simulink model "ICAR"  (R2018b)
settings: Solver=FixedStepAuto  StartTime=0.0  StopTime=10.0  RelTol=1e-3
(part 3 of 4)

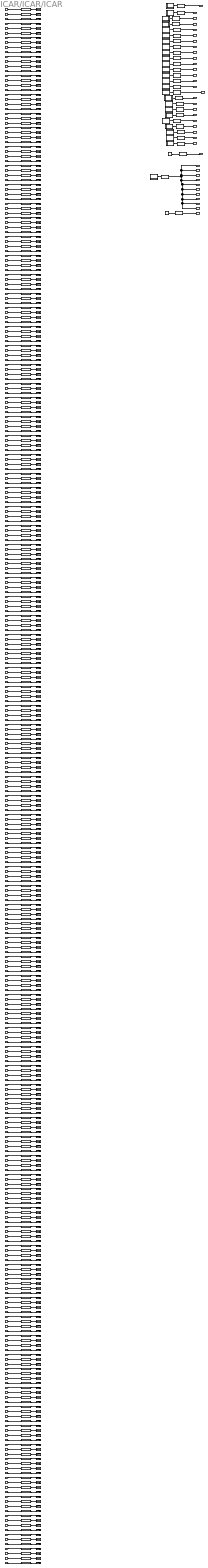
== system ICAR/ICAR/ICAR ==
  System_Clock : Inport  OutDataTypeStr=UInt16
  FDMMve_d_IcaFcnConf : Inport  Port=2  OutDataTypeStr=UInt16
  FDMMve_d_SignalTStamp : Inport  Port=3  OutDataTypeStr=UInt16
  ICABva_g_VehParameter : Inport  Port=4  OutDataTypeStr=T_M_Nm_Float32  PortDimensions=60
  ICABva_g_FilterInfo : Inport  Port=5  OutDataTypeStr=T_M_Nm_Float32  PortDimensions=50
  ICABve_d_SignalTStamp : Inport  Port=6  OutDataTypeStr=UInt16
  IMAPve_d_EPS_LKA_State : Inport  Port=7  OutDataTypeStr=UInt16
  IMAPve_g_EPS_SW_Trq : Inport  Port=8  OutDataTypeStr=T_M_Nm_Float32
  IMAPve_d_EPS_Error_State : Inport  Port=9  OutDataTypeStr=UInt16
  IMAPve_d_EPS_Trq_State : Inport  Port=10  OutDataTypeStr=UInt16
  IMAPve_d_SAS_Clb_State : Inport  Port=11  OutDataTypeStr=UInt16
  IMAPve_d_SAS_Trim_State : Inport  Port=12  OutDataTypeStr=UInt16
  IMAPve_d_EPS_TrqLim_State : Inport  Port=13  OutDataTypeStr=UInt16
  IMAPve_g_EPS_LKA_Current : Inport  Port=14  OutDataTypeStr=T_M_Nm_Float32
  IMAPve_g_ESC_LatAcc : Inport  Port=15  OutDataTypeStr=T_M_Nm_Float32
  IMAPve_d_ESC_LatAcc_Valid : Inport  Port=16  OutDataTypeStr=UInt16
  IMAPve_g_ESC_YawRate : Inport  Port=17  OutDataTypeStr=T_M_Nm_Float32
  IMAPve_d_ESC_YawRate_Valid : Inport  Port=18  OutDataTypeStr=UInt16
  IMAPve_g_ESC_UnYawRate : Inport  Port=19  OutDataTypeStr=T_M_Nm_Float32
  IMAPve_g_ESC_VehSpd : Inport  Port=20  OutDataTypeStr=T_M_Nm_Float32
  IMAPve_g_ESC_LonAcc : Inport  Port=21  OutDataTypeStr=T_M_Nm_Float32
  IMAPve_d_ESC_LonAcc_Valid : Inport  Port=22  OutDataTypeStr=UInt16
  IMAPve_g_ESC_Brake_Press : Inport  Port=23  OutDataTypeStr=T_M_Nm_Float32
  IMAPve_g_ESC_Static_Slope : Inport  Port=24  OutDataTypeStr=T_M_Nm_Float32
  IMAPve_g_ESC_DySlope_Accuracy : Inport  Port=25  OutDataTypeStr=T_M_Nm_Float32
  IMAPve_g_ESC_DySlope : Inport  Port=26  OutDataTypeStr=T_M_Nm_Float32
  IMAPve_g_SW_Angle : Inport  Port=27  OutDataTypeStr=T_M_Nm_Float32
  IMAPve_g_SW_Angle_Speed : Inport  Port=28  OutDataTypeStr=T_M_Nm_Float32
  IMAPve_d_BCM_HazardLamp : Inport  Port=29  OutDataTypeStr=UInt16
  IMAPve_d_BCM_Left_Light : Inport  Port=30  OutDataTypeStr=UInt16
  IMAPve_d_BCM_Right_Light : Inport  Port=31  OutDataTypeStr=UInt16
  IMAPve_d_ESC_BrakeLamp_Req : Inport  Port=32  OutDataTypeStr=UInt16
  IMAPve_d_BCM_Opening_State : Inport  Port=33  OutDataTypeStr=UInt16
  IMAPve_d_BCM_Trunk_State : Inport  Port=34  OutDataTypeStr=UInt16
  IMAPve_d_BCM_LF_Door_State : Inport  Port=35  OutDataTypeStr=UInt16
  IMAPve_d_BCM_RF_Door_State : Inport  Port=36  OutDataTypeStr=UInt16
  IMAPve_d_BCM_RR_Door_State : Inport  Port=37  OutDataTypeStr=UInt16
  IMAPve_d_BCM_LR_Door_State : Inport  Port=38  OutDataTypeStr=UInt16
  IMAPve_d_SCC_Left_SwitchSig : Inport  Port=39  OutDataTypeStr=UInt16
  IMAPve_d_SCC_Right_SwitchSig : Inport  Port=40  OutDataTypeStr=UInt16
  IMAPve_d_PEPS_Door_Lock_Req : Inport  Port=41  OutDataTypeStr=UInt16
  IMAPve_d_BCM_Door_Lock_State : Inport  Port=42  OutDataTypeStr=UInt16
  IMAPve_d_EMS_ACC_Status : Inport  Port=43  OutDataTypeStr=UInt16
  IMAPve_g_EMS_Pot_WhlT_Max : Inport  Port=44  OutDataTypeStr=T_M_Nm_Float32
  IMAPve_g_EMS_Pot_WhlT_Min : Inport  Port=45  OutDataTypeStr=T_M_Nm_Float32
  IMAPve_g_EMS_RealPedal : Inport  Port=46  OutDataTypeStr=T_M_Nm_Float32
  IMAPve_g_EMS_MaxTWhl : Inport  Port=47  OutDataTypeStr=T_M_Nm_Float32
  IMAPve_g_EMS_MaxTWhl_Offset : Inport  Port=48  OutDataTypeStr=T_M_Nm_Float32
  IMAPve_g_EMS_MinTWhl : Inport  Port=49  OutDataTypeStr=T_M_Nm_Float32
  IMAPve_g_EMS_MinTWhl_Offset : Inport  Port=50  OutDataTypeStr=T_M_Nm_Float32
  IMAPve_g_EMS_Actual_FlwT : Inport  Port=51  OutDataTypeStr=T_M_Nm_Float32
  IMAPve_g_EMS_Actual_IndT : Inport  Port=52  OutDataTypeStr=T_M_Nm_Float32
  IMAPve_g_EMS_Realize_TWhl : Inport  Port=53  OutDataTypeStr=T_M_Nm_Float32
  IMAPve_g_EMS_ACC_VirtualPedal : Inport  Port=54  OutDataTypeStr=T_M_Nm_Float32
  IMAPve_d_EMS_AccPedal_Fault : Inport  Port=55  OutDataTypeStr=UInt16
  IMAPve_g_EMS_Driver_Torque : Inport  Port=56  OutDataTypeStr=T_M_Nm_Float32
  IMAPve_d_ESC_Brake_Effort : Inport  Port=57  OutDataTypeStr=UInt16
  IMAPve_g_EMS_Engine_Speed : Inport  Port=58  OutDataTypeStr=T_M_Nm_Float32
  IMAPve_d_ESC_Veh_Standstill : Inport  Port=59  OutDataTypeStr=UInt16
  IMAPve_d_TCU_Actual_Gear : Inport  Port=60  OutDataTypeStr=UInt16
  IMAPve_d_TCU_Target_Gear : Inport  Port=61  OutDataTypeStr=UInt16
  IMAPve_d_TCU_PRND_State : Inport  Port=62  OutDataTypeStr=UInt16
  IMAPve_d_BCM_Ignition_State : Inport  Port=63  OutDataTypeStr=UInt16
  IMAPve_d_ACU_Driver_Belt : Inport  Port=64  OutDataTypeStr=UInt16
  IMAPve_d_SWS_Fault_Code : Inport  Port=65  OutDataTypeStr=UInt16
  IMAPve_d_SWS_Failure_Status : Inport  Port=66  OutDataTypeStr=UInt16
  IMAPve_d_ESC_OFF : Inport  Port=67  OutDataTypeStr=UInt16
  IMAPve_d_ESC_AlarmSig : Inport  Port=68  OutDataTypeStr=UInt16
  IMAPve_d_Speed_Limit_Switch : Inport  Port=69  OutDataTypeStr=UInt16
  IMAPve_d_ESC_ESC_Active : Inport  Port=70  OutDataTypeStr=UInt16
  IMAPve_d_ESC_MSR_Active : Inport  Port=71  OutDataTypeStr=UInt16
  IMAPve_d_ESC_TCS_Active : Inport  Port=72  OutDataTypeStr=UInt16
  IMAPve_d_ESC_VehSpd_Valid : Inport  Port=73  OutDataTypeStr=UInt16
  IMAPve_d_Brake_Pedal_Fault : Inport  Port=74  OutDataTypeStr=UInt16
  IMAPve_d_ESC_ABS_Active : Inport  Port=75  OutDataTypeStr=UInt16
  IMAPve_d_ESC_ABS_Valid : Inport  Port=76  OutDataTypeStr=UInt16
  IMAPve_d_ESC_ABS_AlarmSig : Inport  Port=77  OutDataTypeStr=UInt16
  IMAPve_d_ESC_FL_WheelPulVal : Inport  Port=78  OutDataTypeStr=UInt16
  IMAPve_d_ESC_FR_WheelPulVal : Inport  Port=79  OutDataTypeStr=UInt16
  IMAPve_d_ESC_RL_WheelPulVal : Inport  Port=80  OutDataTypeStr=UInt16
  IMAPve_d_ESC_RR_WheelPulVal : Inport  Port=81  OutDataTypeStr=UInt16
  IMAPve_g_ESC_FL_WhlSpd : Inport  Port=82  OutDataTypeStr=T_M_Nm_Float32
  IMAPve_d_ESC_FL_WhlSpd_Fault : Inport  Port=83  OutDataTypeStr=UInt16
  IMAPve_g_ESC_FR_WhlSpd : Inport  Port=84  OutDataTypeStr=T_M_Nm_Float32
  IMAPve_d_ESC_FR_WhlSpd_Fault : Inport  Port=85  OutDataTypeStr=UInt16
  IMAPve_g_ESC_RL_WhlSpd : Inport  Port=86  OutDataTypeStr=T_M_Nm_Float32
  IMAPve_d_ESC_RL_WhlSpd_Fault : Inport  Port=87  OutDataTypeStr=UInt16
  IMAPve_g_ESC_RR_WhlSpd : Inport  Port=88  OutDataTypeStr=T_M_Nm_Float32
  IMAPve_d_ESC_RR_WhlSpd_Fault : Inport  Port=89  OutDataTypeStr=UInt16
  IMAPve_d_ESC_FL_Wheel_Pulse : Inport  Port=90  OutDataTypeStr=UInt16
  IMAPve_d_ESC_FR_Wheel_Pulse : Inport  Port=91  OutDataTypeStr=UInt16
  IMAPve_d_ESC_RL_Wheel_Pulse : Inport  Port=92  OutDataTypeStr=UInt16
  IMAPve_d_ESC_RR_Wheel_Pulse : Inport  Port=93  OutDataTypeStr=UInt16
  IMAPve_d_TCU_AT_Failure : Inport  Port=94  OutDataTypeStr=UInt16
  IMAPve_d_TCU_Shift_Valid : Inport  Port=95  OutDataTypeStr=UInt16
  IMAPve_d_TCU_DCT_Clutch_State : Inport  Port=96  OutDataTypeStr=UInt16
  IMAPve_d_TCU_Gear_Engage : Inport  Port=97  OutDataTypeStr=UInt16
  IMAPve_d_TCU_Select_ATMode : Inport  Port=98  OutDataTypeStr=UInt16
  IMAPve_d_EMS_Engine_Status : Inport  Port=99  OutDataTypeStr=UInt16
  IMAPve_d_EMS_Gearbox_CtlAvail : Inport  Port=100  OutDataTypeStr=UInt16
  IMAPve_d_ESC_Brake_Failsafe : Inport  Port=101  OutDataTypeStr=UInt16
  IMAPve_d_ESC_AEB_Status : Inport  Port=102  OutDataTypeStr=UInt16
  IMAPve_d_ESC_AEB_Available : Inport  Port=103  OutDataTypeStr=UInt16
  IMAPve_d_ESC_AEB_Active : Inport  Port=104  OutDataTypeStr=UInt16
  IMAPve_d_ESC_ACC_Status : Inport  Port=105  OutDataTypeStr=UInt16
  IMAPve_d_ESC_ACC_Available : Inport  Port=106  OutDataTypeStr=UInt16
  IMAPve_d_ESC_ACC_Active : Inport  Port=107  OutDataTypeStr=UInt16
  IMAPve_d_EMS_ACC_Effective : Inport  Port=108  OutDataTypeStr=UInt16
  IMAPve_d_BCM_FrontWiper_State : Inport  Port=109  OutDataTypeStr=UInt16
  IMAPve_d_BCM_CHMSL_Status : Inport  Port=110  OutDataTypeStr=UInt16
  IMAPve_d_BCM_BrakeLamp_State : Inport  Port=111  OutDataTypeStr=UInt16
  IMAPve_d_GW_Brake_Only_Req : Inport  Port=112  OutDataTypeStr=UInt16
  IMAPve_d_ACU_Passenger_Belt : Inport  Port=113  OutDataTypeStr=UInt16
  IMAPve_d_EMS_ACC_CtlAvail : Inport  Port=114  OutDataTypeStr=UInt16
  IMAPve_d_EMS_ACC_Inhibited : Inport  Port=115  OutDataTypeStr=UInt16
  IMAPve_d_EMS_Brake_Pedal : Inport  Port=116  OutDataTypeStr=UInt16
  IMAPve_d_BCM_LowBeam_State : Inport  Port=117  OutDataTypeStr=UInt16
  IMAPve_d_BCM_HighBeam_State : Inport  Port=118  OutDataTypeStr=UInt16
  IMAPve_d_EPB_Status : Inport  Port=119  OutDataTypeStr=UInt16
  IMAPve_d_EPB_Display_Req : Inport  Port=120  OutDataTypeStr=UInt16
  IMAPve_d_EPB_Warn_Req : Inport  Port=121  OutDataTypeStr=UInt16
  IMAPve_d_EPB_Switch_State : Inport  Port=122  OutDataTypeStr=UInt16
  IMAPve_d_EPB_Switch_Valid : Inport  Port=123  OutDataTypeStr=UInt16
  IMAPve_d_ESC_Drive_Direction : Inport  Port=124  OutDataTypeStr=UInt16
  IMAPve_d_ESC_Hold_State : Inport  Port=125  OutDataTypeStr=UInt16
  IMAPve_d_EPS_Steer_Hold_State : Inport  Port=126  OutDataTypeStr=UInt16
  IMAPve_d_EPS_Warning_State : Inport  Port=127  OutDataTypeStr=UInt16
  IMAPve_g_EPS_PowerCon : Inport  Port=128  OutDataTypeStr=T_M_Nm_Float32
  IMAPve_d_ESC_EBD_AlarmSig : Inport  Port=129  OutDataTypeStr=UInt16
  IMAPve_d_ESC_AVH_Status : Inport  Port=130  OutDataTypeStr=UInt16
  IMAPve_d_Radar_Detective_Req : Inport  Port=131  OutDataTypeStr=UInt16
  IMAPve_g_BCM_Battery_Voltage : Inport  Port=132  OutDataTypeStr=T_M_Nm_Float32
  IMAPve_d_TBOX_LocalTimeY : Inport  Port=133  OutDataTypeStr=UInt16
  IMAPve_d_TBOX_LocalTimeM : Inport  Port=134  OutDataTypeStr=UInt16
  IMAPve_d_TBOX_LocalTimeD : Inport  Port=135  OutDataTypeStr=UInt16
  IMAPve_d_TBOX_LocalTimeH : Inport  Port=136  OutDataTypeStr=UInt16
  IMAPve_d_TBOX_LocalTimeMin : Inport  Port=137  OutDataTypeStr=UInt16
  IMAPve_d_TBOX_LocalTimeS : Inport  Port=138  OutDataTypeStr=UInt16
  IMAPve_d_TBOX_LocalTime_Valid : Inport  Port=139  OutDataTypeStr=UInt16
  IMAPve_d_TPMS_Warn_Indicate : Inport  Port=140  OutDataTypeStr=UInt16
  IMAPve_d_Radar_State : Inport  Port=141  OutDataTypeStr=UInt16
  IMAPve_d_ACC_Desired_Headway : Inport  Port=142  OutDataTypeStr=UInt16
  IMAPve_d_Time_System_Clock : Inport  Port=143  OutDataTypeStr=UInt16
  IMAPve_d_Signal_Time_Stamp : Inport  Port=144  OutDataTypeStr=UInt16
  IMAPve_g_GW_IC_Odometer : Inport  Port=145  OutDataTypeStr=UInt32
  IMAPve_g_FAPA_State : Inport  Port=146  OutDataTypeStr=UInt32
  IMAPve_d_Outside_Temp : Inport  Port=147  OutDataTypeStr=UInt16
  IMAPve_d_ORI_CIPV_ID : Inport  Port=148  OutDataTypeStr=UInt16
  IMAPve_d_ORI_Obj_Num : Inport  Port=149  OutDataTypeStr=UInt16
  IMAPva_g_ORI_Probability : Inport  Port=150  OutDataTypeStr=T_M_Nm_Float32  PortDimensions=16
  IMAPva_d_ORI_Obj_Class : Inport  Port=151  OutDataTypeStr=UInt16  PortDimensions=16
  IMAPva_d_ORI_Obj_Motion : Inport  Port=152  OutDataTypeStr=UInt16  PortDimensions=16
  IMAPva_g_ORI_Obj_RelVel : Inport  Port=153  OutDataTypeStr=T_M_Nm_Float32  PortDimensions=16
  IMAPva_g_ORI_Obj_LongDis : Inport  Port=154  OutDataTypeStr=T_M_Nm_Float32  PortDimensions=16
  IMAPva_d_ORI_Obj_Lane : Inport  Port=155  OutDataTypeStr=UInt16  PortDimensions=16
  IMAPva_g_ORI_Obj_LAngle : Inport  Port=156  OutDataTypeStr=T_M_Nm_Float32  PortDimensions=16
  IMAPva_g_ORI_Obj_RAngle : Inport  Port=157  OutDataTypeStr=T_M_Nm_Float32  PortDimensions=16
  IMAPva_g_ORI_Obj_Width : Inport  Port=158  OutDataTypeStr=T_M_Nm_Float32  PortDimensions=16
  IMAPva_d_ORI_Obj_ID : Inport  Port=159  OutDataTypeStr=UInt16  PortDimensions=16
  IMAPve_d_ORI_Lane_Valid : Inport  Port=160  OutDataTypeStr=UInt16
  IMAPve_d_ORI_Lane_ConsArea : Inport  Port=161  OutDataTypeStr=UInt16
  IMAPve_d_ORI_Lane_RoadType : Inport  Port=162  OutDataTypeStr=UInt16
  IMAPve_g_ORI_L0_C3 : Inport  Port=163  OutDataTypeStr=T_M_Nm_Float32
  IMAPve_g_ORI_L0_C2 : Inport  Port=164  OutDataTypeStr=T_M_Nm_Float32
  IMAPve_g_ORI_L0_C1 : Inport  Port=165  OutDataTypeStr=T_M_Nm_Float32
  IMAPve_g_ORI_L0_C0 : Inport  Port=166  OutDataTypeStr=T_M_Nm_Float32
  IMAPve_d_ORI_L0_Q : Inport  Port=167  OutDataTypeStr=UInt16
  IMAPve_d_ORI_L0_Type : Inport  Port=168  OutDataTypeStr=UInt16
  IMAPve_g_ORI_L0_VR : Inport  Port=169  OutDataTypeStr=T_M_Nm_Float32
  IMAPve_g_ORI_L0_TLC : Inport  Port=170  OutDataTypeStr=T_M_Nm_Float32
  IMAPve_g_ORI_L0_W : Inport  Port=171  OutDataTypeStr=T_M_Nm_Float32
  IMAPve_d_ORI_L0_LC : Inport  Port=172  OutDataTypeStr=UInt16
  IMAPve_g_ORI_L1_C3 : Inport  Port=173  OutDataTypeStr=T_M_Nm_Float32
  IMAPve_g_ORI_L1_C2 : Inport  Port=174  OutDataTypeStr=T_M_Nm_Float32
  IMAPve_g_ORI_L1_C1 : Inport  Port=175  OutDataTypeStr=T_M_Nm_Float32
  IMAPve_g_ORI_L1_C0 : Inport  Port=176  OutDataTypeStr=T_M_Nm_Float32
  IMAPve_d_ORI_L1_Q : Inport  Port=177  OutDataTypeStr=UInt16
  IMAPve_d_ORI_L1_Type : Inport  Port=178  OutDataTypeStr=UInt16
  IMAPve_g_ORI_L1_VR : Inport  Port=179  OutDataTypeStr=T_M_Nm_Float32
  IMAPve_g_ORI_L1_TLC : Inport  Port=180  OutDataTypeStr=T_M_Nm_Float32
  IMAPve_g_ORI_L1_W : Inport  Port=181  OutDataTypeStr=T_M_Nm_Float32
  IMAPve_d_ORI_L1_LC : Inport  Port=182  OutDataTypeStr=UInt16
  IMAPve_g_ORI_R0_C3 : Inport  Port=183  OutDataTypeStr=T_M_Nm_Float32
  IMAPve_g_ORI_R0_C2 : Inport  Port=184  OutDataTypeStr=T_M_Nm_Float32
  IMAPve_g_ORI_R0_C1 : Inport  Port=185  OutDataTypeStr=T_M_Nm_Float32
  IMAPve_g_ORI_R0_C0 : Inport  Port=186  OutDataTypeStr=T_M_Nm_Float32
  IMAPve_d_ORI_R0_Q : Inport  Port=187  OutDataTypeStr=UInt16
  IMAPve_d_ORI_R0_LT : Inport  Port=188  OutDataTypeStr=UInt16
  IMAPve_g_ORI_R0_VR : Inport  Port=189  OutDataTypeStr=T_M_Nm_Float32
  IMAPve_g_ORI_R0_TLC : Inport  Port=190  OutDataTypeStr=T_M_Nm_Float32
  IMAPve_g_ORI_R0_W : Inport  Port=191  OutDataTypeStr=T_M_Nm_Float32
  IMAPve_d_ORI_R0_LC : Inport  Port=192  OutDataTypeStr=UInt16
  IMAPve_g_ORI_R1_C3 : Inport  Port=193  OutDataTypeStr=T_M_Nm_Float32
  IMAPve_g_ORI_R1_C2 : Inport  Port=194  OutDataTypeStr=T_M_Nm_Float32
  IMAPve_g_ORI_R1_C1 : Inport  Port=195  OutDataTypeStr=T_M_Nm_Float32
  IMAPve_g_ORI_R1_C0 : Inport  Port=196  OutDataTypeStr=T_M_Nm_Float32
  IMAPve_d_ORI_R1_Q : Inport  Port=197  OutDataTypeStr=UInt16
  IMAPve_d_ORI_R1_LT : Inport  Port=198  OutDataTypeStr=UInt16
  IMAPve_g_ORI_R1_VR : Inport  Port=199  OutDataTypeStr=T_M_Nm_Float32
  IMAPve_g_ORI_R1_TLC : Inport  Port=200  OutDataTypeStr=T_M_Nm_Float32
  IMAPve_g_ORI_R1_W : Inport  Port=201  OutDataTypeStr=T_M_Nm_Float32
  IMAPve_d_ORI_R1_LC : Inport  Port=202  OutDataTypeStr=UInt16
  IMAPve_d_Sensor_Status : Inport  Port=203  OutDataTypeStr=UInt16
  IMAPve_d_LF_Radar_Status : Inport  Port=204  OutDataTypeStr=UInt16
  IMAPve_d_RF_Radar_Status : Inport  Port=205  OutDataTypeStr=UInt16
  IMAPve_d_LR_Radar_Status : Inport  Port=206  OutDataTypeStr=UInt16
  IMAPve_d_RR_Radar_Status : Inport  Port=207  OutDataTypeStr=UInt16
  IMAPve_d_Fusion_Status : Inport  Port=208  OutDataTypeStr=UInt16
  IMAPve_g_Fusion_Time_Stamp : Inport  Port=209  OutDataTypeStr=T_M_Nm_Float32
  IMAPve_d_obj_Num : Inport  Port=210  OutDataTypeStr=UInt16
  IMAPva_d_obj_id : Inport  Port=211  OutDataTypeStr=UInt16  PortDimensions=40
  IMAPva_g_obj_pos_x : Inport  Port=212  OutDataTypeStr=T_M_Nm_Float32  PortDimensions=40
  IMAPva_g_obj_pos_y : Inport  Port=213  OutDataTypeStr=T_M_Nm_Float32  PortDimensions=40
  IMAPva_g_obj_vel_x : Inport  Port=214  OutDataTypeStr=T_M_Nm_Float32  PortDimensions=40
  IMAPva_g_obj_vel_y : Inport  Port=215  OutDataTypeStr=T_M_Nm_Float32  PortDimensions=40
  IMAPva_g_obj_acc_x : Inport  Port=216  OutDataTypeStr=T_M_Nm_Float32  PortDimensions=40
  IMAPva_g_obj_acc_y : Inport  Port=217  OutDataTypeStr=T_M_Nm_Float32  PortDimensions=40
  IMAPva_g_obj_pos_var_x : Inport  Port=218  OutDataTypeStr=T_M_Nm_Float32  PortDimensions=40
  IMAPva_g_obj_pos_var_y : Inport  Port=219  OutDataTypeStr=T_M_Nm_Float32  PortDimensions=40
  IMAPva_g_obj_pos_var_xy : Inport  Port=220  OutDataTypeStr=T_M_Nm_Float32  PortDimensions=40
  IMAPva_g_obj_vel_var_x : Inport  Port=221  OutDataTypeStr=T_M_Nm_Float32  PortDimensions=40
  IMAPva_g_obj_vel_var_y : Inport  Port=222  OutDataTypeStr=T_M_Nm_Float32  PortDimensions=40
  IMAPva_g_obj_vel_var_xy : Inport  Port=223  OutDataTypeStr=T_M_Nm_Float32  PortDimensions=40
  IMAPva_g_obj_width : Inport  Port=224  OutDataTypeStr=T_M_Nm_Float32  PortDimensions=40
  IMAPva_g_obj_length : Inport  Port=225  OutDataTypeStr=T_M_Nm_Float32  PortDimensions=40
  IMAPva_d_obj_fusion_type : Inport  Port=226  OutDataTypeStr=UInt16  PortDimensions=40
  IMAPva_d_obj_class : Inport  Port=227  OutDataTypeStr=UInt16  PortDimensions=40
  IMAPva_d_obj_lane : Inport  Port=228  OutDataTypeStr=UInt16  PortDimensions=40
  IMAPva_d_obj_status : Inport  Port=229  OutDataTypeStr=UInt16  PortDimensions=40
  IMAPva_d_obj_cam_asso_id : Inport  Port=230  OutDataTypeStr=UInt16  PortDimensions=40
  IMAPva_g_obj_con : Inport  Port=231  OutDataTypeStr=T_M_Nm_Float32  PortDimensions=40
  IMAPva_g_obj_age : Inport  Port=232  OutDataTypeStr=T_M_Nm_Float32  PortDimensions=40
  IMAPva_d_obj_TurnLight : Inport  Port=233  OutDataTypeStr=UInt16  PortDimensions=40
  IMAPva_d_obj_BrakeLight : Inport  Port=234  OutDataTypeStr=UInt16  PortDimensions=40
  IMAPva_d_obj_MotionStatus : Inport  Port=235  OutDataTypeStr=UInt16  PortDimensions=40
  IMAPva_d_obj_ACC : Inport  Port=236  OutDataTypeStr=UInt16  PortDimensions=40
  IMAPva_d_obj_AEB : Inport  Port=237  OutDataTypeStr=UInt16  PortDimensions=40
  IMAPva_d_obj_ELK : Inport  Port=238  OutDataTypeStr=UInt16  PortDimensions=40
  IMAPva_d_obj_ALC : Inport  Port=239  OutDataTypeStr=UInt16  PortDimensions=40
  IMAPva_d_obj_ESA : Inport  Port=240  OutDataTypeStr=UInt16  PortDimensions=40
  IMAPva_d_obj_JA : Inport  Port=241  OutDataTypeStr=UInt16  PortDimensions=40
  IMAPve_d_Lane_Valid : Inport  Port=242  OutDataTypeStr=UInt16
  IMAPve_d_Road_Type : Inport  Port=243  OutDataTypeStr=UInt16
  IMAPve_d_ConsArea : Inport  Port=244  OutDataTypeStr=UInt16
  IMAPve_g_L0_C0 : Inport  Port=245  OutDataTypeStr=T_M_Nm_Float32
  IMAPve_g_L0_C1 : Inport  Port=246  OutDataTypeStr=T_M_Nm_Float32
  IMAPve_g_L0_C2 : Inport  Port=247  OutDataTypeStr=T_M_Nm_Float32
  IMAPve_g_L0_C3 : Inport  Port=248  OutDataTypeStr=T_M_Nm_Float32
  IMAPve_g_L0_VR : Inport  Port=249  OutDataTypeStr=T_M_Nm_Float32
  IMAPve_d_L0_Q : Inport  Port=250  OutDataTypeStr=UInt16
  IMAPve_d_L0_Type : Inport  Port=251  OutDataTypeStr=UInt16
  IMAPve_g_L0_Confidence : Inport  Port=252  OutDataTypeStr=T_M_Nm_Float32
  IMAPve_g_L0_W : Inport  Port=253  OutDataTypeStr=T_M_Nm_Float32
  IMAPve_g_L0_TLC : Inport  Port=254  OutDataTypeStr=T_M_Nm_Float32
  IMAPve_d_L0_LC : Inport  Port=255  OutDataTypeStr=UInt16
  IMAPve_g_R0_C0 : Inport  Port=256  OutDataTypeStr=T_M_Nm_Float32
  IMAPve_g_R0_C1 : Inport  Port=257  OutDataTypeStr=T_M_Nm_Float32
  IMAPve_g_R0_C2 : Inport  Port=258  OutDataTypeStr=T_M_Nm_Float32
  IMAPve_g_R0_C3 : Inport  Port=259  OutDataTypeStr=T_M_Nm_Float32
  IMAPve_g_R0_VR : Inport  Port=260  OutDataTypeStr=T_M_Nm_Float32
  IMAPve_d_R0_Q : Inport  Port=261  OutDataTypeStr=UInt16
  IMAPve_d_R0_Type : Inport  Port=262  OutDataTypeStr=UInt16
  IMAPve_g_R0_Confidence : Inport  Port=263  OutDataTypeStr=T_M_Nm_Float32
  IMAPve_g_R0_W : Inport  Port=264  OutDataTypeStr=T_M_Nm_Float32
  IMAPve_g_R0_TLC : Inport  Port=265  OutDataTypeStr=T_M_Nm_Float32
  IMAPve_d_R0_LC : Inport  Port=266  OutDataTypeStr=UInt16
  IMAPve_g_L1_C0 : Inport  Port=267  OutDataTypeStr=T_M_Nm_Float32
  IMAPve_g_L1_C1 : Inport  Port=268  OutDataTypeStr=T_M_Nm_Float32
  IMAPve_g_L1_C2 : Inport  Port=269  OutDataTypeStr=T_M_Nm_Float32
  IMAPve_g_L1_C3 : Inport  Port=270  OutDataTypeStr=T_M_Nm_Float32
  IMAPve_g_L1_VR : Inport  Port=271  OutDataTypeStr=T_M_Nm_Float32
  IMAPve_d_L1_Q : Inport  Port=272  OutDataTypeStr=UInt16
  IMAPve_d_L1_Type : Inport  Port=273  OutDataTypeStr=UInt16
  IMAPve_g_L1_Confidence : Inport  Port=274  OutDataTypeStr=T_M_Nm_Float32
  IMAPve_g_L1_W : Inport  Port=275  OutDataTypeStr=T_M_Nm_Float32
  IMAPve_g_L1_TLC : Inport  Port=276  OutDataTypeStr=T_M_Nm_Float32
  IMAPve_d_L1_LC : Inport  Port=277  OutDataTypeStr=UInt16
  IMAPve_g_R1_C0 : Inport  Port=278  OutDataTypeStr=T_M_Nm_Float32
  IMAPve_g_R1_C1 : Inport  Port=279  OutDataTypeStr=T_M_Nm_Float32
  IMAPve_g_R1_C2 : Inport  Port=280  OutDataTypeStr=T_M_Nm_Float32
  IMAPve_g_R1_C3 : Inport  Port=281  OutDataTypeStr=T_M_Nm_Float32
  IMAPve_g_R1_VR : Inport  Port=282  OutDataTypeStr=T_M_Nm_Float32
  IMAPve_d_R1_Q : Inport  Port=283  OutDataTypeStr=UInt16
  IMAPve_d_R1_Type : Inport  Port=284  OutDataTypeStr=UInt16
  IMAPve_g_R1_Confidence : Inport  Port=285  OutDataTypeStr=T_M_Nm_Float32
  IMAPve_g_R1_W : Inport  Port=286  OutDataTypeStr=T_M_Nm_Float32
  IMAPve_g_R1_TLC : Inport  Port=287  OutDataTypeStr=T_M_Nm_Float32
  IMAPve_d_R1_LC : Inport  Port=288  OutDataTypeStr=UInt16
  IMAPve_g_L0_C0_Back : Inport  Port=289  OutDataTypeStr=T_M_Nm_Float32
  IMAPve_g_L0_C1_Back : Inport  Port=290  OutDataTypeStr=T_M_Nm_Float32
  IMAPve_g_L0_C2_Back : Inport  Port=291  OutDataTypeStr=T_M_Nm_Float32
  IMAPve_g_L0_C3_Back : Inport  Port=292  OutDataTypeStr=T_M_Nm_Float32
  IMAPve_g_L0_Range_Back : Inport  Port=293  OutDataTypeStr=T_M_Nm_Float32
  IMAPve_g_L0_C0_FR_Pred : Inport  Port=294  OutDataTypeStr=T_M_Nm_Float32
  IMAPve_g_L0_C1_FR_Pred : Inport  Port=295  OutDataTypeStr=T_M_Nm_Float32
  IMAPve_g_L0_C2_FR_Pred : Inport  Port=296  OutDataTypeStr=T_M_Nm_Float32
  IMAPve_g_L0_Range_FR_Pred : Inport  Port=297  OutDataTypeStr=T_M_Nm_Float32
  IMAPve_g_R0_C0_Back : Inport  Port=298  OutDataTypeStr=T_M_Nm_Float32
  IMAPve_g_R0_C1_Back : Inport  Port=299  OutDataTypeStr=T_M_Nm_Float32
  IMAPve_g_R0_C2_Back : Inport  Port=300  OutDataTypeStr=T_M_Nm_Float32
  IMAPve_g_R0_C3_Back : Inport  Port=301  OutDataTypeStr=T_M_Nm_Float32
  IMAPve_g_R0_Range_Back : Inport  Port=302  OutDataTypeStr=T_M_Nm_Float32
  IMAPve_g_R0_C0_FR_Pred : Inport  Port=303  OutDataTypeStr=T_M_Nm_Float32
  IMAPve_g_R0_C1_FR_Pred : Inport  Port=304  OutDataTypeStr=T_M_Nm_Float32
  IMAPve_g_R0_C2_FR_Pred : Inport  Port=305  OutDataTypeStr=T_M_Nm_Float32
  IMAPve_g_R0_Range_FR_Pred : Inport  Port=306  OutDataTypeStr=T_M_Nm_Float32
  IMAPve_g_L1_C0_Back : Inport  Port=307  OutDataTypeStr=T_M_Nm_Float32
  IMAPve_g_L1_C1_Back : Inport  Port=308  OutDataTypeStr=T_M_Nm_Float32
  IMAPve_g_L1_C2_Back : Inport  Port=309  OutDataTypeStr=T_M_Nm_Float32
  IMAPve_g_L1_C3_Back : Inport  Port=310  OutDataTypeStr=T_M_Nm_Float32
  IMAPve_g_L1_Range_Back : Inport  Port=311  OutDataTypeStr=T_M_Nm_Float32
  IMAPve_g_L1_C0_FR_Pred : Inport  Port=312  OutDataTypeStr=T_M_Nm_Float32
  IMAPve_g_L1_C1_FR_Pred : Inport  Port=313  OutDataTypeStr=T_M_Nm_Float32
  IMAPve_g_L1_C2_FR_Pred : Inport  Port=314  OutDataTypeStr=T_M_Nm_Float32
  IMAPve_g_L1_Range_FR_Pred : Inport  Port=315  OutDataTypeStr=T_M_Nm_Float32
  IMAPve_g_R1_C0_Back : Inport  Port=316  OutDataTypeStr=T_M_Nm_Float32
  IMAPve_g_R1_C1_Back : Inport  Port=317  OutDataTypeStr=T_M_Nm_Float32
  IMAPve_g_R1_C2_Back : Inport  Port=318  OutDataTypeStr=T_M_Nm_Float32
  IMAPve_g_R1_C3_Back : Inport  Port=319  OutDataTypeStr=T_M_Nm_Float32
  IMAPve_g_R1_Range_Back : Inport  Port=320  OutDataTypeStr=T_M_Nm_Float32
  IMAPve_g_R1_C0_FR_Pred : Inport  Port=321  OutDataTypeStr=T_M_Nm_Float32
  IMAPve_g_R1_C1_FR_Pred : Inport  Port=322  OutDataTypeStr=T_M_Nm_Float32
  IMAPve_g_R1_C2_FR_Pred : Inport  Port=323  OutDataTypeStr=T_M_Nm_Float32
  IMAPve_g_R1_Range_FR_Pred : Inport  Port=324  OutDataTypeStr=T_M_Nm_Float32
  IMAPve_d_Sign_ISA_Value : Inport  Port=325  OutDataTypeStr=UInt16
  IMAPve_d_TSR_Sign_Type : Inport  Port=326  OutDataTypeStr=UInt16
  IMAPve_d_Camera_Signal_Fault : Inport  Port=327  OutDataTypeStr=UInt16
  IMAPve_d_Radar_Status : Inport  Port=328  OutDataTypeStr=UInt16
  IMAPve_d_Camera_Status : Inport  Port=329  OutDataTypeStr=UInt16
  Constant : Constant
  Constant1 : Constant
  Data Type Conversion{,2,14..27} (16 alike) : DataTypeConversion  OutDataTypeStr=T_M_Nm_Float32
  Data Type Conversion{1,3..13} (12 alike) : DataTypeConversion  OutDataTypeStr=UInt16
  FDMMve_d_IcaFcnConf_1 : Terminator
  FDMMve_d_IcaFcnConf_convert : DataTypeConversion  OutDataTypeStr=uint8
  FDMMve_d_SignalTStamp_1 : Terminator
  FDMMve_d_SignalTStamp_convert : DataTypeConversion  OutDataTypeStr=uint8
  ICABva_g_FilterInfo_1 : Terminator
  ICABva_g_FilterInfo_convert : DataTypeConversion  OutDataTypeStr=uint8
  ICABva_g_VehParameter_1 : Terminator
  ICABva_g_VehParameter_convert : DataTypeConversion  OutDataTypeStr=uint8
  ICABve_d_SignalTStamp_1 : Terminator
  ICABve_d_SignalTStamp_convert : DataTypeConversion  OutDataTypeStr=uint8
  IMAPva_d_ORI_Obj_Class_1 : Terminator
  IMAPva_d_ORI_Obj_Class_convert : DataTypeConversion  OutDataTypeStr=uint8
  IMAPva_d_ORI_Obj_ID_1 : Terminator
  IMAPva_d_ORI_Obj_ID_convert : DataTypeConversion  OutDataTypeStr=uint8
  IMAPva_d_ORI_Obj_Lane_1 : Terminator
  IMAPva_d_ORI_Obj_Lane_convert : DataTypeConversion  OutDataTypeStr=uint8
  IMAPva_d_ORI_Obj_Motion_1 : Terminator
  IMAPva_d_ORI_Obj_Motion_convert : DataTypeConversion  OutDataTypeStr=uint8
  IMAPva_d_obj_ACC_1 : Terminator
  IMAPva_d_obj_ACC_convert : DataTypeConversion  OutDataTypeStr=uint8
  IMAPva_d_obj_AEB_1 : Terminator
  IMAPva_d_obj_AEB_convert : DataTypeConversion  OutDataTypeStr=uint8
  IMAPva_d_obj_ALC_1 : Terminator
  IMAPva_d_obj_ALC_convert : DataTypeConversion  OutDataTypeStr=uint8
  IMAPva_d_obj_BrakeLight_1 : Terminator
  IMAPva_d_obj_BrakeLight_convert : DataTypeConversion  OutDataTypeStr=uint8
  IMAPva_d_obj_ELK_1 : Terminator
  IMAPva_d_obj_ELK_convert : DataTypeConversion  OutDataTypeStr=uint8
  IMAPva_d_obj_ESA_1 : Terminator
  IMAPva_d_obj_ESA_convert : DataTypeConversion  OutDataTypeStr=uint8
  IMAPva_d_obj_JA_1 : Terminator
  IMAPva_d_obj_JA_convert : DataTypeConversion  OutDataTypeStr=uint8
  IMAPva_d_obj_MotionStatus_1 : Terminator
  IMAPva_d_obj_MotionStatus_convert : DataTypeConversion  OutDataTypeStr=uint8
  IMAPva_d_obj_TurnLight_1 : Terminator
  IMAPva_d_obj_TurnLight_convert : DataTypeConversion  OutDataTypeStr=uint8
  IMAPva_d_obj_cam_asso_id_1 : Terminator
  IMAPva_d_obj_cam_asso_id_convert : DataTypeConversion  OutDataTypeStr=uint8
  IMAPva_d_obj_class_1 : Terminator
  IMAPva_d_obj_class_convert : DataTypeConversion  OutDataTypeStr=uint8
  IMAPva_d_obj_fusion_type_1 : Terminator
  IMAPva_d_obj_fusion_type_convert : DataTypeConversion  OutDataTypeStr=uint8
  IMAPva_d_obj_id_1 : Terminator
  IMAPva_d_obj_id_convert : DataTypeConversion  OutDataTypeStr=uint8
  IMAPva_d_obj_lane_1 : Terminator
  IMAPva_d_obj_lane_convert : DataTypeConversion  OutDataTypeStr=uint8
  IMAPva_d_obj_status_1 : Terminator
  IMAPva_d_obj_status_convert : DataTypeConversion  OutDataTypeStr=uint8
  IMAPva_g_ORI_Obj_LAngle_1 : Terminator
  IMAPva_g_ORI_Obj_LAngle_convert : DataTypeConversion  OutDataTypeStr=uint8
  IMAPva_g_ORI_Obj_LongDis_1 : Terminator
  IMAPva_g_ORI_Obj_LongDis_convert : DataTypeConversion  OutDataTypeStr=uint8
  IMAPva_g_ORI_Obj_RAngle_1 : Terminator
  IMAPva_g_ORI_Obj_RAngle_convert : DataTypeConversion  OutDataTypeStr=uint8
  IMAPva_g_ORI_Obj_RelVel_1 : Terminator
  IMAPva_g_ORI_Obj_RelVel_convert : DataTypeConversion  OutDataTypeStr=uint8
  IMAPva_g_ORI_Obj_Width_1 : Terminator
  IMAPva_g_ORI_Obj_Width_convert : DataTypeConversion  OutDataTypeStr=uint8
  IMAPva_g_ORI_Probability_1 : Terminator
  IMAPva_g_ORI_Probability_convert : DataTypeConversion  OutDataTypeStr=uint8
  IMAPva_g_obj_acc_x_1 : Terminator
  IMAPva_g_obj_acc_x_convert : DataTypeConversion  OutDataTypeStr=uint8
  IMAPva_g_obj_acc_y_1 : Terminator
  IMAPva_g_obj_acc_y_convert : DataTypeConversion  OutDataTypeStr=uint8
  IMAPva_g_obj_age_1 : Terminator
  IMAPva_g_obj_age_convert : DataTypeConversion  OutDataTypeStr=uint8
  IMAPva_g_obj_con_1 : Terminator
  IMAPva_g_obj_con_convert : DataTypeConversion  OutDataTypeStr=uint8
  IMAPva_g_obj_length_1 : Terminator
  IMAPva_g_obj_length_convert : DataTypeConversion  OutDataTypeStr=uint8
  IMAPva_g_obj_pos_var_x_1 : Terminator
  IMAPva_g_obj_pos_var_x_convert : DataTypeConversion  OutDataTypeStr=uint8
  IMAPva_g_obj_pos_var_xy_1 : Terminator
  IMAPva_g_obj_pos_var_xy_convert : DataTypeConversion  OutDataTypeStr=uint8
  IMAPva_g_obj_pos_var_y_1 : Terminator
  IMAPva_g_obj_pos_var_y_convert : DataTypeConversion  OutDataTypeStr=uint8
  IMAPva_g_obj_pos_x_1 : Terminator
  IMAPva_g_obj_pos_x_convert : DataTypeConversion  OutDataTypeStr=uint8
  IMAPva_g_obj_pos_y_1 : Terminator
  IMAPva_g_obj_pos_y_convert : DataTypeConversion  OutDataTypeStr=uint8
  IMAPva_g_obj_vel_var_x_1 : Terminator
  IMAPva_g_obj_vel_var_x_convert : DataTypeConversion  OutDataTypeStr=uint8
  IMAPva_g_obj_vel_var_xy_1 : Terminator
  IMAPva_g_obj_vel_var_xy_convert : DataTypeConversion  OutDataTypeStr=uint8
  IMAPva_g_obj_vel_var_y_1 : Terminator
  IMAPva_g_obj_vel_var_y_convert : DataTypeConversion  OutDataTypeStr=uint8
  IMAPva_g_obj_vel_x_1 : Terminator
  IMAPva_g_obj_vel_x_convert : DataTypeConversion  OutDataTypeStr=uint8
  IMAPva_g_obj_vel_y_1 : Terminator
  IMAPva_g_obj_vel_y_convert : DataTypeConversion  OutDataTypeStr=uint8
  IMAPva_g_obj_width_1 : Terminator
  IMAPva_g_obj_width_convert : DataTypeConversion  OutDataTypeStr=uint8
  IMAPve_d_ACC_Desired_Headway_1 : Terminator
  IMAPve_d_ACC_Desired_Headway_convert : DataTypeConversion  OutDataTypeStr=uint8
  IMAPve_d_ACU_Driver_Belt_1 : Terminator
  IMAPve_d_ACU_Driver_Belt_convert : DataTypeConversion  OutDataTypeStr=uint8
  IMAPve_d_ACU_Passenger_Belt_1 : Terminator
  IMAPve_d_ACU_Passenger_Belt_convert : DataTypeConversion  OutDataTypeStr=uint8
  IMAPve_d_BCM_BrakeLamp_State_1 : Terminator
  IMAPve_d_BCM_BrakeLamp_State_convert : DataTypeConversion  OutDataTypeStr=uint8
  IMAPve_d_BCM_CHMSL_Status_1 : Terminator
  IMAPve_d_BCM_CHMSL_Status_convert : DataTypeConversion  OutDataTypeStr=uint8
  IMAPve_d_BCM_Door_Lock_State_1 : Terminator
  IMAPve_d_BCM_Door_Lock_State_convert : DataTypeConversion  OutDataTypeStr=uint8
  IMAPve_d_BCM_FrontWiper_State_1 : Terminator
  IMAPve_d_BCM_FrontWiper_State_convert : DataTypeConversion  OutDataTypeStr=uint8
  IMAPve_d_BCM_HazardLamp_1 : Terminator
  IMAPve_d_BCM_HazardLamp_convert : DataTypeConversion  OutDataTypeStr=uint8
  IMAPve_d_BCM_HighBeam_State_1 : Terminator
  IMAPve_d_BCM_HighBeam_State_convert : DataTypeConversion  OutDataTypeStr=uint8
  IMAPve_d_BCM_Ignition_State_1 : Terminator
  IMAPve_d_BCM_Ignition_State_convert : DataTypeConversion  OutDataTypeStr=uint8
  IMAPve_d_BCM_LF_Door_State_1 : Terminator
  IMAPve_d_BCM_LF_Door_State_convert : DataTypeConversion  OutDataTypeStr=uint8
  IMAPve_d_BCM_LR_Door_State_1 : Terminator
  IMAPve_d_BCM_LR_Door_State_convert : DataTypeConversion  OutDataTypeStr=uint8
  IMAPve_d_BCM_Left_Light_1 : Terminator
  IMAPve_d_BCM_Left_Light_convert : DataTypeConversion  OutDataTypeStr=uint8
  IMAPve_d_BCM_LowBeam_State_1 : Terminator
  IMAPve_d_BCM_LowBeam_State_convert : DataTypeConversion  OutDataTypeStr=uint8
  IMAPve_d_BCM_Opening_State_1 : Terminator
  IMAPve_d_BCM_Opening_State_convert : DataTypeConversion  OutDataTypeStr=uint8
  IMAPve_d_BCM_RF_Door_State_1 : Terminator
  IMAPve_d_BCM_RF_Door_State_convert : DataTypeConversion  OutDataTypeStr=uint8
  IMAPve_d_BCM_RR_Door_State_1 : Terminator
  IMAPve_d_BCM_RR_Door_State_convert : DataTypeConversion  OutDataTypeStr=uint8
  IMAPve_d_BCM_Right_Light_1 : Terminator
  IMAPve_d_BCM_Right_Light_convert : DataTypeConversion  OutDataTypeStr=uint8
  IMAPve_d_BCM_Trunk_State_1 : Terminator
  IMAPve_d_BCM_Trunk_State_convert : DataTypeConversion  OutDataTypeStr=uint8
  IMAPve_d_Brake_Pedal_Fault_1 : Terminator
  IMAPve_d_Brake_Pedal_Fault_convert : DataTypeConversion  OutDataTypeStr=uint8
  IMAPve_d_Camera_Signal_Fault_1 : Terminator
  IMAPve_d_Camera_Signal_Fault_convert : DataTypeConversion  OutDataTypeStr=uint8
  IMAPve_d_Camera_Status_1 : Terminator
  IMAPve_d_Camera_Status_convert : DataTypeConversion  OutDataTypeStr=uint8
  IMAPve_d_ConsArea_1 : Terminator
  IMAPve_d_ConsArea_convert : DataTypeConversion  OutDataTypeStr=uint8
  IMAPve_d_EMS_ACC_CtlAvail_1 : Terminator
  IMAPve_d_EMS_ACC_CtlAvail_convert : DataTypeConversion  OutDataTypeStr=uint8
  IMAPve_d_EMS_ACC_Effective_1 : Terminator
  IMAPve_d_EMS_ACC_Effective_convert : DataTypeConversion  OutDataTypeStr=uint8
  IMAPve_d_EMS_ACC_Inhibited_1 : Terminator
  IMAPve_d_EMS_ACC_Inhibited_convert : DataTypeConversion  OutDataTypeStr=uint8
  IMAPve_d_EMS_ACC_Status_1 : Terminator
  IMAPve_d_EMS_ACC_Status_convert : DataTypeConversion  OutDataTypeStr=uint8
  IMAPve_d_EMS_AccPedal_Fault_1 : Terminator
  IMAPve_d_EMS_AccPedal_Fault_convert : DataTypeConversion  OutDataTypeStr=uint8
  IMAPve_d_EMS_Brake_Pedal_1 : Terminator
  IMAPve_d_EMS_Brake_Pedal_convert : DataTypeConversion  OutDataTypeStr=uint8
  IMAPve_d_EMS_Engine_Status_1 : Terminator
  IMAPve_d_EMS_Engine_Status_convert : DataTypeConversion  OutDataTypeStr=uint8
  IMAPve_d_EMS_Gearbox_CtlAvail_1 : Terminator
  IMAPve_d_EMS_Gearbox_CtlAvail_convert : DataTypeConversion  OutDataTypeStr=uint8
  IMAPve_d_EPB_Display_Req_1 : Terminator
  IMAPve_d_EPB_Display_Req_convert : DataTypeConversion  OutDataTypeStr=uint8
  IMAPve_d_EPB_Status_1 : Terminator
  IMAPve_d_EPB_Status_convert : DataTypeConversion  OutDataTypeStr=uint8
  IMAPve_d_EPB_Switch_State_1 : Terminator
  IMAPve_d_EPB_Switch_State_convert : DataTypeConversion  OutDataTypeStr=uint8
  IMAPve_d_EPB_Switch_Valid_1 : Terminator
  IMAPve_d_EPB_Switch_Valid_convert : DataTypeConversion  OutDataTypeStr=uint8
  IMAPve_d_EPB_Warn_Req_1 : Terminator
  IMAPve_d_EPB_Warn_Req_convert : DataTypeConversion  OutDataTypeStr=uint8
  IMAPve_d_EPS_Error_State_1 : Terminator
  IMAPve_d_EPS_Error_State_convert : DataTypeConversion  OutDataTypeStr=uint8
  IMAPve_d_EPS_LKA_State_1 : Terminator
  IMAPve_d_EPS_LKA_State_convert : DataTypeConversion  OutDataTypeStr=uint8
  IMAPve_d_EPS_Steer_Hold_State_1 : Terminator
  IMAPve_d_EPS_Steer_Hold_State_convert : DataTypeConversion  OutDataTypeStr=uint8
  IMAPve_d_EPS_TrqLim_State_1 : Terminator
  IMAPve_d_EPS_TrqLim_State_convert : DataTypeConversion  OutDataTypeStr=uint8
  IMAPve_d_EPS_Trq_State_1 : Terminator
  IMAPve_d_EPS_Trq_State_convert : DataTypeConversion  OutDataTypeStr=uint8
  IMAPve_d_EPS_Warning_State_1 : Terminator
  IMAPve_d_EPS_Warning_State_convert : DataTypeConversion  OutDataTypeStr=uint8
  IMAPve_d_ESC_ABS_Active_1 : Terminator
  IMAPve_d_ESC_ABS_Active_convert : DataTypeConversion  OutDataTypeStr=uint8
  IMAPve_d_ESC_ABS_AlarmSig_1 : Terminator
  IMAPve_d_ESC_ABS_AlarmSig_convert : DataTypeConversion  OutDataTypeStr=uint8
  IMAPve_d_ESC_ABS_Valid_1 : Terminator
  IMAPve_d_ESC_ABS_Valid_convert : DataTypeConversion  OutDataTypeStr=uint8
  IMAPve_d_ESC_ACC_Active_1 : Terminator
  IMAPve_d_ESC_ACC_Active_convert : DataTypeConversion  OutDataTypeStr=uint8
  IMAPve_d_ESC_ACC_Available_1 : Terminator
  IMAPve_d_ESC_ACC_Available_convert : DataTypeConversion  OutDataTypeStr=uint8
  IMAPve_d_ESC_ACC_Status_1 : Terminator
  IMAPve_d_ESC_ACC_Status_convert : DataTypeConversion  OutDataTypeStr=uint8
  IMAPve_d_ESC_AEB_Active_1 : Terminator
  IMAPve_d_ESC_AEB_Active_convert : DataTypeConversion  OutDataTypeStr=uint8
  IMAPve_d_ESC_AEB_Available_1 : Terminator
  IMAPve_d_ESC_AEB_Available_convert : DataTypeConversion  OutDataTypeStr=uint8
  IMAPve_d_ESC_AEB_Status_1 : Terminator
  IMAPve_d_ESC_AEB_Status_convert : DataTypeConversion  OutDataTypeStr=uint8
  IMAPve_d_ESC_AVH_Status_1 : Terminator
  IMAPve_d_ESC_AVH_Status_convert : DataTypeConversion  OutDataTypeStr=uint8
  IMAPve_d_ESC_AlarmSig_1 : Terminator
  IMAPve_d_ESC_AlarmSig_convert : DataTypeConversion  OutDataTypeStr=uint8
  IMAPve_d_ESC_BrakeLamp_Req_1 : Terminator
  IMAPve_d_ESC_BrakeLamp_Req_convert : DataTypeConversion  OutDataTypeStr=uint8
  IMAPve_d_ESC_Brake_Effort_1 : Terminator
  IMAPve_d_ESC_Brake_Effort_convert : DataTypeConversion  OutDataTypeStr=uint8
  IMAPve_d_ESC_Brake_Failsafe_1 : Terminator
  IMAPve_d_ESC_Brake_Failsafe_convert : DataTypeConversion  OutDataTypeStr=uint8
  IMAPve_d_ESC_Drive_Direction_1 : Terminator
  IMAPve_d_ESC_Drive_Direction_convert : DataTypeConversion  OutDataTypeStr=uint8
  IMAPve_d_ESC_EBD_AlarmSig_1 : Terminator
  IMAPve_d_ESC_EBD_AlarmSig_convert : DataTypeConversion  OutDataTypeStr=uint8
  IMAPve_d_ESC_ESC_Active_1 : Terminator
  IMAPve_d_ESC_ESC_Active_convert : DataTypeConversion  OutDataTypeStr=uint8
  IMAPve_d_ESC_FL_WheelPulVal_1 : Terminator
  IMAPve_d_ESC_FL_WheelPulVal_convert : DataTypeConversion  OutDataTypeStr=uint8
  IMAPve_d_ESC_FL_Wheel_Pulse_1 : Terminator
  IMAPve_d_ESC_FL_Wheel_Pulse_convert : DataTypeConversion  OutDataTypeStr=uint8
  IMAPve_d_ESC_FL_WhlSpd_Fault_1 : Terminator
  IMAPve_d_ESC_FL_WhlSpd_Fault_convert : DataTypeConversion  OutDataTypeStr=uint8
  IMAPve_d_ESC_FR_WheelPulVal_1 : Terminator
  IMAPve_d_ESC_FR_WheelPulVal_convert : DataTypeConversion  OutDataTypeStr=uint8
  IMAPve_d_ESC_FR_Wheel_Pulse_1 : Terminator
  IMAPve_d_ESC_FR_Wheel_Pulse_convert : DataTypeConversion  OutDataTypeStr=uint8
  IMAPve_d_ESC_FR_WhlSpd_Fault_1 : Terminator
  IMAPve_d_ESC_FR_WhlSpd_Fault_convert : DataTypeConversion  OutDataTypeStr=uint8
  IMAPve_d_ESC_Hold_State_1 : Terminator
  IMAPve_d_ESC_Hold_State_convert : DataTypeConversion  OutDataTypeStr=uint8
  IMAPve_d_ESC_LatAcc_Valid_1 : Terminator
  IMAPve_d_ESC_LatAcc_Valid_convert : DataTypeConversion  OutDataTypeStr=uint8
  IMAPve_d_ESC_LonAcc_Valid_1 : Terminator
  IMAPve_d_ESC_LonAcc_Valid_convert : DataTypeConversion  OutDataTypeStr=uint8
  IMAPve_d_ESC_MSR_Active_1 : Terminator
  IMAPve_d_ESC_MSR_Active_convert : DataTypeConversion  OutDataTypeStr=uint8
  IMAPve_d_ESC_OFF_1 : Terminator
  IMAPve_d_ESC_OFF_convert : DataTypeConversion  OutDataTypeStr=uint8
  IMAPve_d_ESC_RL_WheelPulVal_1 : Terminator
  IMAPve_d_ESC_RL_WheelPulVal_convert : DataTypeConversion  OutDataTypeStr=uint8
  IMAPve_d_ESC_RL_Wheel_Pulse_1 : Terminator
  IMAPve_d_ESC_RL_Wheel_Pulse_convert : DataTypeConversion  OutDataTypeStr=uint8
  IMAPve_d_ESC_RL_WhlSpd_Fault_1 : Terminator
  IMAPve_d_ESC_RL_WhlSpd_Fault_convert : DataTypeConversion  OutDataTypeStr=uint8
  IMAPve_d_ESC_RR_WheelPulVal_1 : Terminator
  IMAPve_d_ESC_RR_WheelPulVal_convert : DataTypeConversion  OutDataTypeStr=uint8
  IMAPve_d_ESC_RR_Wheel_Pulse_1 : Terminator
  IMAPve_d_ESC_RR_Wheel_Pulse_convert : DataTypeConversion  OutDataTypeStr=uint8
  IMAPve_d_ESC_RR_WhlSpd_Fault_1 : Terminator
  IMAPve_d_ESC_RR_WhlSpd_Fault_convert : DataTypeConversion  OutDataTypeStr=uint8
  IMAPve_d_ESC_TCS_Active_1 : Terminator
  IMAPve_d_ESC_TCS_Active_convert : DataTypeConversion  OutDataTypeStr=uint8
  IMAPve_d_ESC_VehSpd_Valid_1 : Terminator
  IMAPve_d_ESC_VehSpd_Valid_convert : DataTypeConversion  OutDataTypeStr=uint8
  IMAPve_d_ESC_Veh_Standstill_1 : Terminator
  IMAPve_d_ESC_Veh_Standstill_convert : DataTypeConversion  OutDataTypeStr=uint8
  IMAPve_d_ESC_YawRate_Valid_1 : Terminator
  IMAPve_d_ESC_YawRate_Valid_convert : DataTypeConversion  OutDataTypeStr=uint8
  IMAPve_d_Fusion_Status_1 : Terminator
  IMAPve_d_Fusion_Status_convert : DataTypeConversion  OutDataTypeStr=uint8
  IMAPve_d_GW_Brake_Only_Req_1 : Terminator
  IMAPve_d_GW_Brake_Only_Req_convert : DataTypeConversion  OutDataTypeStr=uint8
  IMAPve_d_L0_LC_1 : Terminator
  IMAPve_d_L0_LC_convert : DataTypeConversion  OutDataTypeStr=uint8
  IMAPve_d_L0_Q_1 : Terminator
  IMAPve_d_L0_Q_convert : DataTypeConversion  OutDataTypeStr=uint8
  IMAPve_d_L0_Type_1 : Terminator
  IMAPve_d_L0_Type_convert : DataTypeConversion  OutDataTypeStr=uint8
  IMAPve_d_L1_LC_1 : Terminator
  IMAPve_d_L1_LC_convert : DataTypeConversion  OutDataTypeStr=uint8
  IMAPve_d_L1_Q_1 : Terminator
  IMAPve_d_L1_Q_convert : DataTypeConversion  OutDataTypeStr=uint8
  IMAPve_d_L1_Type_1 : Terminator
  IMAPve_d_L1_Type_convert : DataTypeConversion  OutDataTypeStr=uint8
  IMAPve_d_LF_Radar_Status_1 : Terminator
  IMAPve_d_LF_Radar_Status_convert : DataTypeConversion  OutDataTypeStr=uint8
  IMAPve_d_LR_Radar_Status_1 : Terminator
  IMAPve_d_LR_Radar_Status_convert : DataTypeConversion  OutDataTypeStr=uint8
  IMAPve_d_Lane_Valid_1 : Terminator
  IMAPve_d_Lane_Valid_convert : DataTypeConversion  OutDataTypeStr=uint8
  IMAPve_d_ORI_CIPV_ID_1 : Terminator
  IMAPve_d_ORI_CIPV_ID_convert : DataTypeConversion  OutDataTypeStr=uint8
  IMAPve_d_ORI_L0_LC_1 : Terminator
  IMAPve_d_ORI_L0_LC_convert : DataTypeConversion  OutDataTypeStr=uint8
  IMAPve_d_ORI_L0_Q_1 : Terminator
  IMAPve_d_ORI_L0_Q_convert : DataTypeConversion  OutDataTypeStr=uint8
  IMAPve_d_ORI_L0_Type_1 : Terminator
  IMAPve_d_ORI_L0_Type_convert : DataTypeConversion  OutDataTypeStr=uint8
  IMAPve_d_ORI_L1_LC_1 : Terminator
  IMAPve_d_ORI_L1_LC_convert : DataTypeConversion  OutDataTypeStr=uint8
  IMAPve_d_ORI_L1_Q_1 : Terminator
  IMAPve_d_ORI_L1_Q_convert : DataTypeConversion  OutDataTypeStr=uint8
  IMAPve_d_ORI_L1_Type_1 : Terminator
  IMAPve_d_ORI_L1_Type_convert : DataTypeConversion  OutDataTypeStr=uint8
  IMAPve_d_ORI_Lane_ConsArea_1 : Terminator
  IMAPve_d_ORI_Lane_ConsArea_convert : DataTypeConversion  OutDataTypeStr=uint8
  IMAPve_d_ORI_Lane_RoadType_1 : Terminator
  IMAPve_d_ORI_Lane_RoadType_convert : DataTypeConversion  OutDataTypeStr=uint8
  IMAPve_d_ORI_Lane_Valid_1 : Terminator
  IMAPve_d_ORI_Lane_Valid_convert : DataTypeConversion  OutDataTypeStr=uint8
  IMAPve_d_ORI_Obj_Num_1 : Terminator
  IMAPve_d_ORI_Obj_Num_convert : DataTypeConversion  OutDataTypeStr=uint8
  IMAPve_d_ORI_R0_LC_1 : Terminator
  IMAPve_d_ORI_R0_LC_convert : DataTypeConversion  OutDataTypeStr=uint8
  IMAPve_d_ORI_R0_LT_1 : Terminator
  IMAPve_d_ORI_R0_LT_convert : DataTypeConversion  OutDataTypeStr=uint8
  IMAPve_d_ORI_R0_Q_1 : Terminator
  IMAPve_d_ORI_R0_Q_convert : DataTypeConversion  OutDataTypeStr=uint8
  IMAPve_d_ORI_R1_LC_1 : Terminator
  IMAPve_d_ORI_R1_LC_convert : DataTypeConversion  OutDataTypeStr=uint8
  IMAPve_d_ORI_R1_LT_1 : Terminator
  IMAPve_d_ORI_R1_LT_convert : DataTypeConversion  OutDataTypeStr=uint8
  IMAPve_d_ORI_R1_Q_1 : Terminator
  IMAPve_d_ORI_R1_Q_convert : DataTypeConversion  OutDataTypeStr=uint8
  IMAPve_d_Outside_Temp_1 : Terminator
  IMAPve_d_Outside_Temp_convert : DataTypeConversion  OutDataTypeStr=uint8
  IMAPve_d_PEPS_Door_Lock_Req_1 : Terminator
  IMAPve_d_PEPS_Door_Lock_Req_convert : DataTypeConversion  OutDataTypeStr=uint8
  IMAPve_d_R0_LC_1 : Terminator
  IMAPve_d_R0_LC_convert : DataTypeConversion  OutDataTypeStr=uint8
  IMAPve_d_R0_Q_1 : Terminator
  IMAPve_d_R0_Q_convert : DataTypeConversion  OutDataTypeStr=uint8
  IMAPve_d_R0_Type_1 : Terminator
  IMAPve_d_R0_Type_convert : DataTypeConversion  OutDataTypeStr=uint8
  IMAPve_d_R1_LC_1 : Terminator
  IMAPve_d_R1_LC_convert : DataTypeConversion  OutDataTypeStr=uint8
  IMAPve_d_R1_Q_1 : Terminator
  IMAPve_d_R1_Q_convert : DataTypeConversion  OutDataTypeStr=uint8
  IMAPve_d_R1_Type_1 : Terminator
  IMAPve_d_R1_Type_convert : DataTypeConversion  OutDataTypeStr=uint8
  IMAPve_d_RF_Radar_Status_1 : Terminator
  IMAPve_d_RF_Radar_Status_convert : DataTypeConversion  OutDataTypeStr=uint8
  IMAPve_d_RR_Radar_Status_1 : Terminator
  IMAPve_d_RR_Radar_Status_convert : DataTypeConversion  OutDataTypeStr=uint8
  IMAPve_d_Radar_Detective_Req_1 : Terminator
  IMAPve_d_Radar_Detective_Req_convert : DataTypeConversion  OutDataTypeStr=uint8
  IMAPve_d_Radar_State_1 : Terminator
  IMAPve_d_Radar_State_convert : DataTypeConversion  OutDataTypeStr=uint8
  IMAPve_d_Radar_Status_1 : Terminator
  IMAPve_d_Radar_Status_convert : DataTypeConversion  OutDataTypeStr=uint8
  IMAPve_d_Road_Type_1 : Terminator
  IMAPve_d_Road_Type_convert : DataTypeConversion  OutDataTypeStr=uint8
  IMAPve_d_SAS_Clb_State_1 : Terminator
  IMAPve_d_SAS_Clb_State_convert : DataTypeConversion  OutDataTypeStr=uint8
  IMAPve_d_SAS_Trim_State_1 : Terminator
  IMAPve_d_SAS_Trim_State_convert : DataTypeConversion  OutDataTypeStr=uint8
  IMAPve_d_SCC_Left_SwitchSig_1 : Terminator
  IMAPve_d_SCC_Left_SwitchSig_convert : DataTypeConversion  OutDataTypeStr=uint8
  IMAPve_d_SCC_Right_SwitchSig_1 : Terminator
  IMAPve_d_SCC_Right_SwitchSig_convert : DataTypeConversion  OutDataTypeStr=uint8
  IMAPve_d_SWS_Failure_Status_1 : Terminator
  IMAPve_d_SWS_Failure_Status_convert : DataTypeConversion  OutDataTypeStr=uint8
  IMAPve_d_SWS_Fault_Code_1 : Terminator
  IMAPve_d_SWS_Fault_Code_convert : DataTypeConversion  OutDataTypeStr=uint8
  IMAPve_d_Sensor_Status_1 : Terminator
  IMAPve_d_Sensor_Status_convert : DataTypeConversion  OutDataTypeStr=uint8
  IMAPve_d_Sign_ISA_Value_1 : Terminator
  IMAPve_d_Sign_ISA_Value_convert : DataTypeConversion  OutDataTypeStr=uint8
  IMAPve_d_Signal_Time_Stamp_1 : Terminator
  IMAPve_d_Signal_Time_Stamp_convert : DataTypeConversion  OutDataTypeStr=uint8
  IMAPve_d_Speed_Limit_Switch_1 : Terminator
  IMAPve_d_Speed_Limit_Switch_convert : DataTypeConversion  OutDataTypeStr=uint8
  IMAPve_d_TBOX_LocalTimeD_1 : Terminator
  IMAPve_d_TBOX_LocalTimeD_convert : DataTypeConversion  OutDataTypeStr=uint8
  IMAPve_d_TBOX_LocalTimeH_1 : Terminator
  IMAPve_d_TBOX_LocalTimeH_convert : DataTypeConversion  OutDataTypeStr=uint8
  IMAPve_d_TBOX_LocalTimeM_1 : Terminator
  IMAPve_d_TBOX_LocalTimeM_convert : DataTypeConversion  OutDataTypeStr=uint8
  IMAPve_d_TBOX_LocalTimeMin_1 : Terminator
  IMAPve_d_TBOX_LocalTimeMin_convert : DataTypeConversion  OutDataTypeStr=uint8
  IMAPve_d_TBOX_LocalTimeS_1 : Terminator
  IMAPve_d_TBOX_LocalTimeS_convert : DataTypeConversion  OutDataTypeStr=uint8
  IMAPve_d_TBOX_LocalTimeY_1 : Terminator
  IMAPve_d_TBOX_LocalTimeY_convert : DataTypeConversion  OutDataTypeStr=uint8
  IMAPve_d_TBOX_LocalTime_Valid_1 : Terminator
  IMAPve_d_TBOX_LocalTime_Valid_convert : DataTypeConversion  OutDataTypeStr=uint8
  IMAPve_d_TCU_AT_Failure_1 : Terminator
  IMAPve_d_TCU_AT_Failure_convert : DataTypeConversion  OutDataTypeStr=uint8
  IMAPve_d_TCU_Actual_Gear_1 : Terminator
  IMAPve_d_TCU_Actual_Gear_convert : DataTypeConversion  OutDataTypeStr=uint8
  IMAPve_d_TCU_DCT_Clutch_State_1 : Terminator
  IMAPve_d_TCU_DCT_Clutch_State_convert : DataTypeConversion  OutDataTypeStr=uint8
  IMAPve_d_TCU_Gear_Engage_1 : Terminator
  IMAPve_d_TCU_Gear_Engage_convert : DataTypeConversion  OutDataTypeStr=uint8
  IMAPve_d_TCU_PRND_State_1 : Terminator
  IMAPve_d_TCU_PRND_State_convert : DataTypeConversion  OutDataTypeStr=uint8
  IMAPve_d_TCU_Select_ATMode_1 : Terminator
  IMAPve_d_TCU_Select_ATMode_convert : DataTypeConversion  OutDataTypeStr=uint8
  IMAPve_d_TCU_Shift_Valid_1 : Terminator
  IMAPve_d_TCU_Shift_Valid_convert : DataTypeConversion  OutDataTypeStr=uint8
  IMAPve_d_TCU_Target_Gear_1 : Terminator
  IMAPve_d_TCU_Target_Gear_convert : DataTypeConversion  OutDataTypeStr=uint8
  IMAPve_d_TPMS_Warn_Indicate_1 : Terminator
  IMAPve_d_TPMS_Warn_Indicate_convert : DataTypeConversion  OutDataTypeStr=uint8
  IMAPve_d_TSR_Sign_Type_1 : Terminator
  IMAPve_d_TSR_Sign_Type_convert : DataTypeConversion  OutDataTypeStr=uint8
  IMAPve_d_Time_System_Clock_1 : Terminator
  IMAPve_d_Time_System_Clock_convert : DataTypeConversion  OutDataTypeStr=uint8
  IMAPve_d_obj_Num_1 : Terminator
  IMAPve_d_obj_Num_convert : DataTypeConversion  OutDataTypeStr=uint8
  IMAPve_g_BCM_Battery_Voltage_1 : Terminator
  IMAPve_g_BCM_Battery_Voltage_convert : DataTypeConversion  OutDataTypeStr=uint8
  IMAPve_g_EMS_ACC_VirtualPedal_1 : Terminator
  IMAPve_g_EMS_ACC_VirtualPedal_convert : DataTypeConversion  OutDataTypeStr=uint8
  IMAPve_g_EMS_Actual_FlwT_1 : Terminator
  IMAPve_g_EMS_Actual_FlwT_convert : DataTypeConversion  OutDataTypeStr=uint8
  IMAPve_g_EMS_Actual_IndT_1 : Terminator
  IMAPve_g_EMS_Actual_IndT_convert : DataTypeConversion  OutDataTypeStr=uint8
  IMAPve_g_EMS_Driver_Torque_1 : Terminator
  IMAPve_g_EMS_Driver_Torque_convert : DataTypeConversion  OutDataTypeStr=uint8
  IMAPve_g_EMS_Engine_Speed_1 : Terminator
  IMAPve_g_EMS_Engine_Speed_convert : DataTypeConversion  OutDataTypeStr=uint8
  IMAPve_g_EMS_MaxTWhl_1 : Terminator
  IMAPve_g_EMS_MaxTWhl_Offset_1 : Terminator
  IMAPve_g_EMS_MaxTWhl_Offset_convert : DataTypeConversion  OutDataTypeStr=uint8
  IMAPve_g_EMS_MaxTWhl_convert : DataTypeConversion  OutDataTypeStr=uint8
  IMAPve_g_EMS_MinTWhl_1 : Terminator
  IMAPve_g_EMS_MinTWhl_Offset_1 : Terminator
  IMAPve_g_EMS_MinTWhl_Offset_convert : DataTypeConversion  OutDataTypeStr=uint8
  IMAPve_g_EMS_MinTWhl_convert : DataTypeConversion  OutDataTypeStr=uint8
  IMAPve_g_EMS_Pot_WhlT_Max_1 : Terminator
  IMAPve_g_EMS_Pot_WhlT_Max_convert : DataTypeConversion  OutDataTypeStr=uint8
  IMAPve_g_EMS_Pot_WhlT_Min_1 : Terminator
  IMAPve_g_EMS_Pot_WhlT_Min_convert : DataTypeConversion  OutDataTypeStr=uint8
  IMAPve_g_EMS_RealPedal_1 : Terminator
  IMAPve_g_EMS_RealPedal_convert : DataTypeConversion  OutDataTypeStr=uint8
  IMAPve_g_EMS_Realize_TWhl_1 : Terminator
  IMAPve_g_EMS_Realize_TWhl_convert : DataTypeConversion  OutDataTypeStr=uint8
  IMAPve_g_EPS_LKA_Current_1 : Terminator
  IMAPve_g_EPS_LKA_Current_convert : DataTypeConversion  OutDataTypeStr=uint8
  IMAPve_g_EPS_PowerCon_1 : Terminator
  IMAPve_g_EPS_PowerCon_convert : DataTypeConversion  OutDataTypeStr=uint8
  IMAPve_g_EPS_SW_Trq_1 : Terminator
  IMAPve_g_EPS_SW_Trq_convert : DataTypeConversion  OutDataTypeStr=uint8
  IMAPve_g_ESC_Brake_Press_1 : Terminator
  IMAPve_g_ESC_Brake_Press_convert : DataTypeConversion  OutDataTypeStr=uint8
  IMAPve_g_ESC_DySlope_1 : Terminator
  IMAPve_g_ESC_DySlope_Accuracy_1 : Terminator
  IMAPve_g_ESC_DySlope_Accuracy_convert : DataTypeConversion  OutDataTypeStr=uint8
  IMAPve_g_ESC_DySlope_convert : DataTypeConversion  OutDataTypeStr=uint8
  IMAPve_g_ESC_FL_WhlSpd_1 : Terminator
  IMAPve_g_ESC_FL_WhlSpd_convert : DataTypeConversion  OutDataTypeStr=uint8
  IMAPve_g_ESC_FR_WhlSpd_1 : Terminator
  IMAPve_g_ESC_FR_WhlSpd_convert : DataTypeConversion  OutDataTypeStr=uint8
  IMAPve_g_ESC_LatAcc_1 : Terminator
  IMAPve_g_ESC_LatAcc_convert : DataTypeConversion  OutDataTypeStr=uint8
  IMAPve_g_ESC_LonAcc_1 : Terminator
  IMAPve_g_ESC_LonAcc_convert : DataTypeConversion  OutDataTypeStr=uint8
  IMAPve_g_ESC_RL_WhlSpd_1 : Terminator
  IMAPve_g_ESC_RL_WhlSpd_convert : DataTypeConversion  OutDataTypeStr=uint8
  IMAPve_g_ESC_RR_WhlSpd_1 : Terminator
  IMAPve_g_ESC_RR_WhlSpd_convert : DataTypeConversion  OutDataTypeStr=uint8
  IMAPve_g_ESC_Static_Slope_1 : Terminator
  IMAPve_g_ESC_Static_Slope_convert : DataTypeConversion  OutDataTypeStr=uint8
  IMAPve_g_ESC_UnYawRate_1 : Terminator
  IMAPve_g_ESC_UnYawRate_convert : DataTypeConversion  OutDataTypeStr=uint8
  IMAPve_g_ESC_VehSpd_1 : Terminator
  IMAPve_g_ESC_VehSpd_convert : DataTypeConversion  OutDataTypeStr=uint8
  IMAPve_g_ESC_YawRate_1 : Terminator
  IMAPve_g_ESC_YawRate_convert : DataTypeConversion  OutDataTypeStr=uint8
  IMAPve_g_FAPA_State_1 : Terminator
  IMAPve_g_FAPA_State_convert : DataTypeConversion  OutDataTypeStr=uint8
  IMAPve_g_Fusion_Time_Stamp_1 : Terminator
  IMAPve_g_Fusion_Time_Stamp_convert : DataTypeConversion  OutDataTypeStr=uint8
  IMAPve_g_GW_IC_Odometer_1 : Terminator
  IMAPve_g_GW_IC_Odometer_convert : DataTypeConversion  OutDataTypeStr=uint8
  IMAPve_g_L0_C0_1 : Terminator
  IMAPve_g_L0_C0_Back_1 : Terminator
  IMAPve_g_L0_C0_Back_convert : DataTypeConversion  OutDataTypeStr=uint8
  IMAPve_g_L0_C0_FR_Pred_1 : Terminator
  IMAPve_g_L0_C0_FR_Pred_convert : DataTypeConversion  OutDataTypeStr=uint8
  IMAPve_g_L0_C0_convert : DataTypeConversion  OutDataTypeStr=uint8
  IMAPve_g_L0_C1_1 : Terminator
  IMAPve_g_L0_C1_Back_1 : Terminator
  IMAPve_g_L0_C1_Back_convert : DataTypeConversion  OutDataTypeStr=uint8
  IMAPve_g_L0_C1_FR_Pred_1 : Terminator
  IMAPve_g_L0_C1_FR_Pred_convert : DataTypeConversion  OutDataTypeStr=uint8
  IMAPve_g_L0_C1_convert : DataTypeConversion  OutDataTypeStr=uint8
  IMAPve_g_L0_C2_1 : Terminator
  IMAPve_g_L0_C2_Back_1 : Terminator
  IMAPve_g_L0_C2_Back_convert : DataTypeConversion  OutDataTypeStr=uint8
  IMAPve_g_L0_C2_FR_Pred_1 : Terminator
  IMAPve_g_L0_C2_FR_Pred_convert : DataTypeConversion  OutDataTypeStr=uint8
  IMAPve_g_L0_C2_convert : DataTypeConversion  OutDataTypeStr=uint8
  IMAPve_g_L0_C3_1 : Terminator
  IMAPve_g_L0_C3_Back_1 : Terminator
  IMAPve_g_L0_C3_Back_convert : DataTypeConversion  OutDataTypeStr=uint8
  IMAPve_g_L0_C3_convert : DataTypeConversion  OutDataTypeStr=uint8
  IMAPve_g_L0_Confidence_1 : Terminator
  IMAPve_g_L0_Confidence_convert : DataTypeConversion  OutDataTypeStr=uint8
  IMAPve_g_L0_Range_Back_1 : Terminator
  IMAPve_g_L0_Range_Back_convert : DataTypeConversion  OutDataTypeStr=uint8
  IMAPve_g_L0_Range_FR_Pred_1 : Terminator
  IMAPve_g_L0_Range_FR_Pred_convert : DataTypeConversion  OutDataTypeStr=uint8
  IMAPve_g_L0_TLC_1 : Terminator
  IMAPve_g_L0_TLC_convert : DataTypeConversion  OutDataTypeStr=uint8
  IMAPve_g_L0_VR_1 : Terminator
  IMAPve_g_L0_VR_convert : DataTypeConversion  OutDataTypeStr=uint8
  IMAPve_g_L0_W_1 : Terminator
  IMAPve_g_L0_W_convert : DataTypeConversion  OutDataTypeStr=uint8
  IMAPve_g_L1_C0_1 : Terminator
  IMAPve_g_L1_C0_Back_1 : Terminator
  IMAPve_g_L1_C0_Back_convert : DataTypeConversion  OutDataTypeStr=uint8
  IMAPve_g_L1_C0_FR_Pred_1 : Terminator
  IMAPve_g_L1_C0_FR_Pred_convert : DataTypeConversion  OutDataTypeStr=uint8
  IMAPve_g_L1_C0_convert : DataTypeConversion  OutDataTypeStr=uint8
  IMAPve_g_L1_C1_1 : Terminator
  IMAPve_g_L1_C1_Back_1 : Terminator
  IMAPve_g_L1_C1_Back_convert : DataTypeConversion  OutDataTypeStr=uint8
  IMAPve_g_L1_C1_FR_Pred_1 : Terminator
  IMAPve_g_L1_C1_FR_Pred_convert : DataTypeConversion  OutDataTypeStr=uint8
  IMAPve_g_L1_C1_convert : DataTypeConversion  OutDataTypeStr=uint8
  IMAPve_g_L1_C2_1 : Terminator
  IMAPve_g_L1_C2_Back_1 : Terminator
  IMAPve_g_L1_C2_Back_convert : DataTypeConversion  OutDataTypeStr=uint8
  IMAPve_g_L1_C2_FR_Pred_1 : Terminator
  IMAPve_g_L1_C2_FR_Pred_convert : DataTypeConversion  OutDataTypeStr=uint8
  IMAPve_g_L1_C2_convert : DataTypeConversion  OutDataTypeStr=uint8
  IMAPve_g_L1_C3_1 : Terminator
  IMAPve_g_L1_C3_Back_1 : Terminator
  IMAPve_g_L1_C3_Back_convert : DataTypeConversion  OutDataTypeStr=uint8
  IMAPve_g_L1_C3_convert : DataTypeConversion  OutDataTypeStr=uint8
  IMAPve_g_L1_Confidence_1 : Terminator
  IMAPve_g_L1_Confidence_convert : DataTypeConversion  OutDataTypeStr=uint8
  IMAPve_g_L1_Range_Back_1 : Terminator
  IMAPve_g_L1_Range_Back_convert : DataTypeConversion  OutDataTypeStr=uint8
  IMAPve_g_L1_Range_FR_Pred_1 : Terminator
  IMAPve_g_L1_Range_FR_Pred_convert : DataTypeConversion  OutDataTypeStr=uint8
  IMAPve_g_L1_TLC_1 : Terminator
  IMAPve_g_L1_TLC_convert : DataTypeConversion  OutDataTypeStr=uint8
  IMAPve_g_L1_VR_1 : Terminator
  IMAPve_g_L1_VR_convert : DataTypeConversion  OutDataTypeStr=uint8
  IMAPve_g_L1_W_1 : Terminator
  IMAPve_g_L1_W_convert : DataTypeConversion  OutDataTypeStr=uint8
  IMAPve_g_ORI_L0_C0_1 : Terminator
  IMAPve_g_ORI_L0_C0_convert : DataTypeConversion  OutDataTypeStr=uint8
  IMAPve_g_ORI_L0_C1_1 : Terminator
  IMAPve_g_ORI_L0_C1_convert : DataTypeConversion  OutDataTypeStr=uint8
  IMAPve_g_ORI_L0_C2_1 : Terminator
  IMAPve_g_ORI_L0_C2_convert : DataTypeConversion  OutDataTypeStr=uint8
  IMAPve_g_ORI_L0_C3_1 : Terminator
  IMAPve_g_ORI_L0_C3_convert : DataTypeConversion  OutDataTypeStr=uint8
  IMAPve_g_ORI_L0_TLC_1 : Terminator
  IMAPve_g_ORI_L0_TLC_convert : DataTypeConversion  OutDataTypeStr=uint8
  IMAPve_g_ORI_L0_VR_1 : Terminator
  IMAPve_g_ORI_L0_VR_convert : DataTypeConversion  OutDataTypeStr=uint8
  IMAPve_g_ORI_L0_W_1 : Terminator
  IMAPve_g_ORI_L0_W_convert : DataTypeConversion  OutDataTypeStr=uint8
  IMAPve_g_ORI_L1_C0_1 : Terminator
  IMAPve_g_ORI_L1_C0_convert : DataTypeConversion  OutDataTypeStr=uint8
  IMAPve_g_ORI_L1_C1_1 : Terminator
  IMAPve_g_ORI_L1_C1_convert : DataTypeConversion  OutDataTypeStr=uint8
  IMAPve_g_ORI_L1_C2_1 : Terminator
  IMAPve_g_ORI_L1_C2_convert : DataTypeConversion  OutDataTypeStr=uint8
  IMAPve_g_ORI_L1_C3_1 : Terminator
  IMAPve_g_ORI_L1_C3_convert : DataTypeConversion  OutDataTypeStr=uint8
  IMAPve_g_ORI_L1_TLC_1 : Terminator
  IMAPve_g_ORI_L1_TLC_convert : DataTypeConversion  OutDataTypeStr=uint8
  IMAPve_g_ORI_L1_VR_1 : Terminator
  IMAPve_g_ORI_L1_VR_convert : DataTypeConversion  OutDataTypeStr=uint8
  IMAPve_g_ORI_L1_W_1 : Terminator
  IMAPve_g_ORI_L1_W_convert : DataTypeConversion  OutDataTypeStr=uint8
  IMAPve_g_ORI_R0_C0_1 : Terminator
  IMAPve_g_ORI_R0_C0_convert : DataTypeConversion  OutDataTypeStr=uint8
  IMAPve_g_ORI_R0_C1_1 : Terminator
  IMAPve_g_ORI_R0_C1_convert : DataTypeConversion  OutDataTypeStr=uint8
  IMAPve_g_ORI_R0_C2_1 : Terminator
  IMAPve_g_ORI_R0_C2_convert : DataTypeConversion  OutDataTypeStr=uint8
  IMAPve_g_ORI_R0_C3_1 : Terminator
  IMAPve_g_ORI_R0_C3_convert : DataTypeConversion  OutDataTypeStr=uint8
  IMAPve_g_ORI_R0_TLC_1 : Terminator
  IMAPve_g_ORI_R0_TLC_convert : DataTypeConversion  OutDataTypeStr=uint8
  IMAPve_g_ORI_R0_VR_1 : Terminator
  IMAPve_g_ORI_R0_VR_convert : DataTypeConversion  OutDataTypeStr=uint8
  IMAPve_g_ORI_R0_W_1 : Terminator
  IMAPve_g_ORI_R0_W_convert : DataTypeConversion  OutDataTypeStr=uint8
  IMAPve_g_ORI_R1_C0_1 : Terminator
  IMAPve_g_ORI_R1_C0_convert : DataTypeConversion  OutDataTypeStr=uint8
  IMAPve_g_ORI_R1_C1_1 : Terminator
  IMAPve_g_ORI_R1_C1_convert : DataTypeConversion  OutDataTypeStr=uint8
  IMAPve_g_ORI_R1_C2_1 : Terminator
  IMAPve_g_ORI_R1_C2_convert : DataTypeConversion  OutDataTypeStr=uint8
  IMAPve_g_ORI_R1_C3_1 : Terminator
  IMAPve_g_ORI_R1_C3_convert : DataTypeConversion  OutDataTypeStr=uint8
  IMAPve_g_ORI_R1_TLC_1 : Terminator
  IMAPve_g_ORI_R1_TLC_convert : DataTypeConversion  OutDataTypeStr=uint8
  IMAPve_g_ORI_R1_VR_1 : Terminator
  IMAPve_g_ORI_R1_VR_convert : DataTypeConversion  OutDataTypeStr=uint8
  IMAPve_g_ORI_R1_W_1 : Terminator
  IMAPve_g_ORI_R1_W_convert : DataTypeConversion  OutDataTypeStr=uint8
  IMAPve_g_R0_C0_1 : Terminator
  IMAPve_g_R0_C0_Back_1 : Terminator
  IMAPve_g_R0_C0_Back_convert : DataTypeConversion  OutDataTypeStr=uint8
  IMAPve_g_R0_C0_FR_Pred_1 : Terminator
  IMAPve_g_R0_C0_FR_Pred_convert : DataTypeConversion  OutDataTypeStr=uint8
  IMAPve_g_R0_C0_convert : DataTypeConversion  OutDataTypeStr=uint8
  IMAPve_g_R0_C1_1 : Terminator
  IMAPve_g_R0_C1_Back_1 : Terminator
  IMAPve_g_R0_C1_Back_convert : DataTypeConversion  OutDataTypeStr=uint8
  IMAPve_g_R0_C1_FR_Pred_1 : Terminator
  IMAPve_g_R0_C1_FR_Pred_convert : DataTypeConversion  OutDataTypeStr=uint8
  IMAPve_g_R0_C1_convert : DataTypeConversion  OutDataTypeStr=uint8
  IMAPve_g_R0_C2_1 : Terminator
  IMAPve_g_R0_C2_Back_1 : Terminator
  IMAPve_g_R0_C2_Back_convert : DataTypeConversion  OutDataTypeStr=uint8
  IMAPve_g_R0_C2_FR_Pred_1 : Terminator
  IMAPve_g_R0_C2_FR_Pred_convert : DataTypeConversion  OutDataTypeStr=uint8
  IMAPve_g_R0_C2_convert : DataTypeConversion  OutDataTypeStr=uint8
  IMAPve_g_R0_C3_1 : Terminator
  IMAPve_g_R0_C3_Back_1 : Terminator
  IMAPve_g_R0_C3_Back_convert : DataTypeConversion  OutDataTypeStr=uint8
  IMAPve_g_R0_C3_convert : DataTypeConversion  OutDataTypeStr=uint8
  IMAPve_g_R0_Confidence_1 : Terminator
  IMAPve_g_R0_Confidence_convert : DataTypeConversion  OutDataTypeStr=uint8
  IMAPve_g_R0_Range_Back_1 : Terminator
  IMAPve_g_R0_Range_Back_convert : DataTypeConversion  OutDataTypeStr=uint8
  IMAPve_g_R0_Range_FR_Pred_1 : Terminator
  IMAPve_g_R0_Range_FR_Pred_convert : DataTypeConversion  OutDataTypeStr=uint8
  IMAPve_g_R0_TLC_1 : Terminator
  IMAPve_g_R0_TLC_convert : DataTypeConversion  OutDataTypeStr=uint8
  IMAPve_g_R0_VR_1 : Terminator
  IMAPve_g_R0_VR_convert : DataTypeConversion  OutDataTypeStr=uint8
  IMAPve_g_R0_W_1 : Terminator
  IMAPve_g_R0_W_convert : DataTypeConversion  OutDataTypeStr=uint8
  IMAPve_g_R1_C0_1 : Terminator
  IMAPve_g_R1_C0_Back_1 : Terminator
  IMAPve_g_R1_C0_Back_convert : DataTypeConversion  OutDataTypeStr=uint8
  IMAPve_g_R1_C0_FR_Pred_1 : Terminator
  IMAPve_g_R1_C0_FR_Pred_convert : DataTypeConversion  OutDataTypeStr=uint8
  IMAPve_g_R1_C0_convert : DataTypeConversion  OutDataTypeStr=uint8
  IMAPve_g_R1_C1_1 : Terminator
  IMAPve_g_R1_C1_Back_1 : Terminator
  IMAPve_g_R1_C1_Back_convert : DataTypeConversion  OutDataTypeStr=uint8
  IMAPve_g_R1_C1_FR_Pred_1 : Terminator
  IMAPve_g_R1_C1_FR_Pred_convert : DataTypeConversion  OutDataTypeStr=uint8
  IMAPve_g_R1_C1_convert : DataTypeConversion  OutDataTypeStr=uint8
  IMAPve_g_R1_C2_1 : Terminator
  IMAPve_g_R1_C2_Back_1 : Terminator
  IMAPve_g_R1_C2_Back_convert : DataTypeConversion  OutDataTypeStr=uint8
  IMAPve_g_R1_C2_FR_Pred_1 : Terminator
  IMAPve_g_R1_C2_FR_Pred_convert : DataTypeConversion  OutDataTypeStr=uint8
  IMAPve_g_R1_C2_convert : DataTypeConversion  OutDataTypeStr=uint8
  IMAPve_g_R1_C3_1 : Terminator
  IMAPve_g_R1_C3_Back_1 : Terminator
  IMAPve_g_R1_C3_Back_convert : DataTypeConversion  OutDataTypeStr=uint8
  IMAPve_g_R1_C3_convert : DataTypeConversion  OutDataTypeStr=uint8
  IMAPve_g_R1_Confidence_1 : Terminator
  IMAPve_g_R1_Confidence_convert : DataTypeConversion  OutDataTypeStr=uint8
  IMAPve_g_R1_Range_Back_1 : Terminator
  IMAPve_g_R1_Range_Back_convert : DataTypeConversion  OutDataTypeStr=uint8
  IMAPve_g_R1_Range_FR_Pred_1 : Terminator
  IMAPve_g_R1_Range_FR_Pred_convert : DataTypeConversion  OutDataTypeStr=uint8
  IMAPve_g_R1_TLC_1 : Terminator
  IMAPve_g_R1_TLC_convert : DataTypeConversion  OutDataTypeStr=uint8
  IMAPve_g_R1_VR_1 : Terminator
  IMAPve_g_R1_VR_convert : DataTypeConversion  OutDataTypeStr=uint8
  IMAPve_g_R1_W_1 : Terminator
  IMAPve_g_R1_W_convert : DataTypeConversion  OutDataTypeStr=uint8
  IMAPve_g_SW_Angle_1 : Terminator
  IMAPve_g_SW_Angle_Speed_1 : Terminator
  IMAPve_g_SW_Angle_Speed_convert : DataTypeConversion  OutDataTypeStr=uint8
  IMAPve_g_SW_Angle_convert : DataTypeConversion  OutDataTypeStr=uint8
  MATLAB Function : MATLAB Function  TreatAsAtomicUnit=on
  MATLAB Function1 : MATLAB Function  TreatAsAtomicUnit=on
  MATLAB Function10 : MATLAB Function  TreatAsAtomicUnit=on
  MATLAB Function11 : MATLAB Function  TreatAsAtomicUnit=on
  MATLAB Function12 : MATLAB Function  TreatAsAtomicUnit=on
  MATLAB Function13 : MATLAB Function  TreatAsAtomicUnit=on
  MATLAB Function14 : MATLAB Function  TreatAsAtomicUnit=on
  MATLAB Function15 : MATLAB Function  TreatAsAtomicUnit=on
  MATLAB Function16 : MATLAB Function  TreatAsAtomicUnit=on
  MATLAB Function17 : MATLAB Function  TreatAsAtomicUnit=on
  MATLAB Function18 : MATLAB Function  TreatAsAtomicUnit=on
  MATLAB Function19 : MATLAB Function  TreatAsAtomicUnit=on
  MATLAB Function20 : MATLAB Function  TreatAsAtomicUnit=on
  MATLAB Function21 : MATLAB Function  TreatAsAtomicUnit=on
  MATLAB Function22 : MATLAB Function  TreatAsAtomicUnit=on
  MATLAB Function23 : MATLAB Function  TreatAsAtomicUnit=on
  MATLAB Function24 : MATLAB Function  TreatAsAtomicUnit=on
  MATLAB Function25 : MATLAB Function  TreatAsAtomicUnit=on
  MATLAB Function26 : MATLAB Function  TreatAsAtomicUnit=on
  MATLAB Function3 : MATLAB Function  TreatAsAtomicUnit=on
  MATLAB Function4 : MATLAB Function  TreatAsAtomicUnit=on
  MATLAB Function5 : MATLAB Function  TreatAsAtomicUnit=on
  MATLAB Function6 : MATLAB Function  TreatAsAtomicUnit=on
  MATLAB Function7 : MATLAB Function  TreatAsAtomicUnit=on
  MATLAB Function8 : MATLAB Function  TreatAsAtomicUnit=on
  MATLAB Function9 : MATLAB Function  TreatAsAtomicUnit=on
  System_Clock_1 : Terminator
  System_Clock_convert : DataTypeConversion  OutDataTypeStr=uint8
  ICARva_d_obj_Num : Outport  OutDataTypeStr=UInt16  PortDimensions=40
  ICARva_d_obj_id : Outport  Port=2  OutDataTypeStr=UInt16  PortDimensions=40
  ICARva_g_obj_pos_x : Outport  Port=3  OutDataTypeStr=T_M_Nm_Float32  PortDimensions=40
  ICARva_g_obj_pos_y : Outport  Port=4  OutDataTypeStr=T_M_Nm_Float32  PortDimensions=40
  ICARva_g_obj_vel_x : Outport  Port=5  OutDataTypeStr=T_M_Nm_Float32  PortDimensions=40
  ICARva_g_obj_vel_y : Outport  Port=6  OutDataTypeStr=T_M_Nm_Float32  PortDimensions=40
  ICARva_g_obj_acc_x : Outport  Port=7  OutDataTypeStr=T_M_Nm_Float32  PortDimensions=40
  ICARva_g_obj_acc_y : Outport  Port=8  OutDataTypeStr=T_M_Nm_Float32  PortDimensions=40
  ICARva_g_obj_pos_var_x : Outport  Port=9  OutDataTypeStr=T_M_Nm_Float32  PortDimensions=40
  ICARva_g_obj_pos_var_y : Outport  Port=10  OutDataTypeStr=T_M_Nm_Float32  PortDimensions=40
  ICARva_g_obj_pos_var_xy : Outport  Port=11  OutDataTypeStr=T_M_Nm_Float32  PortDimensions=40
  ICARva_g_obj_vel_var_x : Outport  Port=12  OutDataTypeStr=T_M_Nm_Float32  PortDimensions=40
  ICARva_g_obj_vel_var_y : Outport  Port=13  OutDataTypeStr=T_M_Nm_Float32  PortDimensions=40
  ICARva_g_obj_vel_var_xy : Outport  Port=14  OutDataTypeStr=T_M_Nm_Float32  PortDimensions=40
  ICARva_g_obj_width : Outport  Port=15  OutDataTypeStr=T_M_Nm_Float32  PortDimensions=40
  ICARva_d_obj_length : Outport  Port=16  OutDataTypeStr=T_M_Nm_Float32  PortDimensions=40
  ICARva_d_obj_fusion_type : Outport  Port=17  OutDataTypeStr=UInt16  PortDimensions=40
  ICARva_d_obj_class : Outport  Port=18  OutDataTypeStr=UInt16  PortDimensions=40
  ICARva_d_obj_lane : Outport  Port=19  OutDataTypeStr=UInt16  PortDimensions=40
  ICARva_d_obj_status : Outport  Port=20  OutDataTypeStr=UInt16  PortDimensions=40
  ICARve_d_obj_cam_asso_id : Outport  Port=21  OutDataTypeStr=UInt16
  ICARva_g_obj_con : Outport  Port=22  OutDataTypeStr=T_M_Nm_Float32  PortDimensions=40
  ICARva_d_obj_age : Outport  Port=23  OutDataTypeStr=UInt16  PortDimensions=40
  ICARva_d_obj_TurnLi : Outport  Port=24  OutDataTypeStr=UInt16  PortDimensions=40
  ICARva_d_obj_BrkLi : Outport  Port=25  OutDataTypeStr=UInt16  PortDimensions=40
  ICARva_d_obj_MtnStat : Outport  Port=26  OutDataTypeStr=UInt16  PortDimensions=40
  ICARva_g_ObjXPre : Outport  Port=27  OutDataTypeStr=T_M_Nm_Float32  PortDimensions=240
  ICARva_g_ObjYPre : Outport  Port=28  OutDataTypeStr=T_M_Nm_Float32  PortDimensions=240
  ICARva_g_ObjVarXPre : Outport  Port=29  OutDataTypeStr=T_M_Nm_Float32  PortDimensions=240
  ICARva_g_ObjVarYPre : Outport  Port=30  OutDataTypeStr=T_M_Nm_Float32  PortDimensions=240
  ICARva_g_ObjVarXYPre : Outport  Port=31  OutDataTypeStr=T_M_Nm_Float32  PortDimensions=240
  ICARva_g_ObjVelXPre : Outport  Port=32  OutDataTypeStr=T_M_Nm_Float32  PortDimensions=240
  ICARva_g_ObjVelYPre : Outport  Port=33  OutDataTypeStr=T_M_Nm_Float32  PortDimensions=240
  ICARva_g_ObjVelVarXPre : Outport  Port=34  OutDataTypeStr=T_M_Nm_Float32  PortDimensions=240
  ICARva_g_ObjVelVarYPre : Outport  Port=35  OutDataTypeStr=T_M_Nm_Float32  PortDimensions=240
  ICARva_g_ObjVelVarXYPre : Outport  Port=36  OutDataTypeStr=T_M_Nm_Float32  PortDimensions=240
  ICARve_d_SignalTStamp : Outport  Port=37  OutDataTypeStr=UInt16
  wires:
  System_Clock/1 -> System_Clock_convert/1
  System_Clock_convert/1 -> System_Clock_1/1
  FDMMve_d_IcaFcnConf/1 -> FDMMve_d_IcaFcnConf_convert/1
  FDMMve_d_IcaFcnConf_convert/1 -> FDMMve_d_IcaFcnConf_1/1
  FDMMve_d_SignalTStamp/1 -> FDMMve_d_SignalTStamp_convert/1
  FDMMve_d_SignalTStamp_convert/1 -> FDMMve_d_SignalTStamp_1/1
  ICABva_g_VehParameter/1 -> ICABva_g_VehParameter_convert/1
  ICABva_g_VehParameter_convert/1 -> ICABva_g_VehParameter_1/1
  ICABva_g_FilterInfo/1 -> ICABva_g_FilterInfo_convert/1
  ICABva_g_FilterInfo_convert/1 -> ICABva_g_FilterInfo_1/1
  ICABve_d_SignalTStamp/1 -> ICABve_d_SignalTStamp_convert/1
  ICABve_d_SignalTStamp_convert/1 -> ICABve_d_SignalTStamp_1/1
  IMAPve_d_EPS_LKA_State/1 -> IMAPve_d_EPS_LKA_State_convert/1
  IMAPve_d_EPS_LKA_State_convert/1 -> IMAPve_d_EPS_LKA_State_1/1
  IMAPve_g_EPS_SW_Trq/1 -> IMAPve_g_EPS_SW_Trq_convert/1
  IMAPve_g_EPS_SW_Trq_convert/1 -> IMAPve_g_EPS_SW_Trq_1/1
  IMAPve_d_EPS_Error_State/1 -> IMAPve_d_EPS_Error_State_convert/1
  IMAPve_d_EPS_Error_State_convert/1 -> IMAPve_d_EPS_Error_State_1/1
  IMAPve_d_EPS_Trq_State/1 -> IMAPve_d_EPS_Trq_State_convert/1
  IMAPve_d_EPS_Trq_State_convert/1 -> IMAPve_d_EPS_Trq_State_1/1
  IMAPve_d_SAS_Clb_State/1 -> IMAPve_d_SAS_Clb_State_convert/1
  IMAPve_d_SAS_Clb_State_convert/1 -> IMAPve_d_SAS_Clb_State_1/1
  IMAPve_d_SAS_Trim_State/1 -> IMAPve_d_SAS_Trim_State_convert/1
  IMAPve_d_SAS_Trim_State_convert/1 -> IMAPve_d_SAS_Trim_State_1/1
  IMAPve_d_EPS_TrqLim_State/1 -> IMAPve_d_EPS_TrqLim_State_convert/1
  IMAPve_d_EPS_TrqLim_State_convert/1 -> IMAPve_d_EPS_TrqLim_State_1/1
  IMAPve_g_EPS_LKA_Current/1 -> IMAPve_g_EPS_LKA_Current_convert/1
  IMAPve_g_EPS_LKA_Current_convert/1 -> IMAPve_g_EPS_LKA_Current_1/1
  IMAPve_g_ESC_LatAcc/1 -> IMAPve_g_ESC_LatAcc_convert/1
  IMAPve_g_ESC_LatAcc_convert/1 -> IMAPve_g_ESC_LatAcc_1/1
  IMAPve_d_ESC_LatAcc_Valid/1 -> IMAPve_d_ESC_LatAcc_Valid_convert/1
  IMAPve_d_ESC_LatAcc_Valid_convert/1 -> IMAPve_d_ESC_LatAcc_Valid_1/1
  IMAPve_g_ESC_YawRate/1 -> IMAPve_g_ESC_YawRate_convert/1
  IMAPve_g_ESC_YawRate_convert/1 -> IMAPve_g_ESC_YawRate_1/1
  IMAPve_d_ESC_YawRate_Valid/1 -> IMAPve_d_ESC_YawRate_Valid_convert/1
  IMAPve_d_ESC_YawRate_Valid_convert/1 -> IMAPve_d_ESC_YawRate_Valid_1/1
  IMAPve_g_ESC_UnYawRate/1 -> IMAPve_g_ESC_UnYawRate_convert/1
  IMAPve_g_ESC_UnYawRate_convert/1 -> IMAPve_g_ESC_UnYawRate_1/1
  IMAPve_g_ESC_VehSpd/1 -> IMAPve_g_ESC_VehSpd_convert/1
  IMAPve_g_ESC_VehSpd_convert/1 -> IMAPve_g_ESC_VehSpd_1/1
  IMAPve_g_ESC_LonAcc/1 -> IMAPve_g_ESC_LonAcc_convert/1
  IMAPve_g_ESC_LonAcc_convert/1 -> IMAPve_g_ESC_LonAcc_1/1
  IMAPve_d_ESC_LonAcc_Valid/1 -> IMAPve_d_ESC_LonAcc_Valid_convert/1
  IMAPve_d_ESC_LonAcc_Valid_convert/1 -> IMAPve_d_ESC_LonAcc_Valid_1/1
  IMAPve_g_ESC_Brake_Press/1 -> IMAPve_g_ESC_Brake_Press_convert/1
  IMAPve_g_ESC_Brake_Press_convert/1 -> IMAPve_g_ESC_Brake_Press_1/1
  IMAPve_g_ESC_Static_Slope/1 -> IMAPve_g_ESC_Static_Slope_convert/1
  IMAPve_g_ESC_Static_Slope_convert/1 -> IMAPve_g_ESC_Static_Slope_1/1
  IMAPve_g_ESC_DySlope_Accuracy/1 -> IMAPve_g_ESC_DySlope_Accuracy_convert/1
  IMAPve_g_ESC_DySlope_Accuracy_convert/1 -> IMAPve_g_ESC_DySlope_Accuracy_1/1
  IMAPve_g_ESC_DySlope/1 -> IMAPve_g_ESC_DySlope_convert/1
  IMAPve_g_ESC_DySlope_convert/1 -> IMAPve_g_ESC_DySlope_1/1
  IMAPve_g_SW_Angle/1 -> IMAPve_g_SW_Angle_convert/1
  IMAPve_g_SW_Angle_convert/1 -> IMAPve_g_SW_Angle_1/1
  IMAPve_g_SW_Angle_Speed/1 -> IMAPve_g_SW_Angle_Speed_convert/1
  IMAPve_g_SW_Angle_Speed_convert/1 -> IMAPve_g_SW_Angle_Speed_1/1
  IMAPve_d_BCM_HazardLamp/1 -> IMAPve_d_BCM_HazardLamp_convert/1
  IMAPve_d_BCM_HazardLamp_convert/1 -> IMAPve_d_BCM_HazardLamp_1/1
  IMAPve_d_BCM_Left_Light/1 -> IMAPve_d_BCM_Left_Light_convert/1
  IMAPve_d_BCM_Left_Light_convert/1 -> IMAPve_d_BCM_Left_Light_1/1
  IMAPve_d_BCM_Right_Light/1 -> IMAPve_d_BCM_Right_Light_convert/1
  IMAPve_d_BCM_Right_Light_convert/1 -> IMAPve_d_BCM_Right_Light_1/1
  IMAPve_d_ESC_BrakeLamp_Req/1 -> IMAPve_d_ESC_BrakeLamp_Req_convert/1
  IMAPve_d_ESC_BrakeLamp_Req_convert/1 -> IMAPve_d_ESC_BrakeLamp_Req_1/1
  IMAPve_d_BCM_Opening_State/1 -> IMAPve_d_BCM_Opening_State_convert/1
  IMAPve_d_BCM_Opening_State_convert/1 -> IMAPve_d_BCM_Opening_State_1/1
  IMAPve_d_BCM_Trunk_State/1 -> IMAPve_d_BCM_Trunk_State_convert/1
  IMAPve_d_BCM_Trunk_State_convert/1 -> IMAPve_d_BCM_Trunk_State_1/1
  IMAPve_d_BCM_LF_Door_State/1 -> IMAPve_d_BCM_LF_Door_State_convert/1
  IMAPve_d_BCM_LF_Door_State_convert/1 -> IMAPve_d_BCM_LF_Door_State_1/1
  IMAPve_d_BCM_RF_Door_State/1 -> IMAPve_d_BCM_RF_Door_State_convert/1
  IMAPve_d_BCM_RF_Door_State_convert/1 -> IMAPve_d_BCM_RF_Door_State_1/1
  IMAPve_d_BCM_RR_Door_State/1 -> IMAPve_d_BCM_RR_Door_State_convert/1
  IMAPve_d_BCM_RR_Door_State_convert/1 -> IMAPve_d_BCM_RR_Door_State_1/1
  IMAPve_d_BCM_LR_Door_State/1 -> IMAPve_d_BCM_LR_Door_State_convert/1
  IMAPve_d_BCM_LR_Door_State_convert/1 -> IMAPve_d_BCM_LR_Door_State_1/1
  IMAPve_d_SCC_Left_SwitchSig/1 -> IMAPve_d_SCC_Left_SwitchSig_convert/1
  IMAPve_d_SCC_Left_SwitchSig_convert/1 -> IMAPve_d_SCC_Left_SwitchSig_1/1
  IMAPve_d_SCC_Right_SwitchSig/1 -> IMAPve_d_SCC_Right_SwitchSig_convert/1
  IMAPve_d_SCC_Right_SwitchSig_convert/1 -> IMAPve_d_SCC_Right_SwitchSig_1/1
  IMAPve_d_PEPS_Door_Lock_Req/1 -> IMAPve_d_PEPS_Door_Lock_Req_convert/1
  IMAPve_d_PEPS_Door_Lock_Req_convert/1 -> IMAPve_d_PEPS_Door_Lock_Req_1/1
  IMAPve_d_BCM_Door_Lock_State/1 -> IMAPve_d_BCM_Door_Lock_State_convert/1
  IMAPve_d_BCM_Door_Lock_State_convert/1 -> IMAPve_d_BCM_Door_Lock_State_1/1
  IMAPve_d_EMS_ACC_Status/1 -> IMAPve_d_EMS_ACC_Status_convert/1
  IMAPve_d_EMS_ACC_Status_convert/1 -> IMAPve_d_EMS_ACC_Status_1/1
  IMAPve_g_EMS_Pot_WhlT_Max/1 -> IMAPve_g_EMS_Pot_WhlT_Max_convert/1
  IMAPve_g_EMS_Pot_WhlT_Max_convert/1 -> IMAPve_g_EMS_Pot_WhlT_Max_1/1
  IMAPve_g_EMS_Pot_WhlT_Min/1 -> IMAPve_g_EMS_Pot_WhlT_Min_convert/1
  IMAPve_g_EMS_Pot_WhlT_Min_convert/1 -> IMAPve_g_EMS_Pot_WhlT_Min_1/1
  IMAPve_g_EMS_RealPedal/1 -> IMAPve_g_EMS_RealPedal_convert/1
  IMAPve_g_EMS_RealPedal_convert/1 -> IMAPve_g_EMS_RealPedal_1/1
  IMAPve_g_EMS_MaxTWhl/1 -> IMAPve_g_EMS_MaxTWhl_convert/1
  IMAPve_g_EMS_MaxTWhl_convert/1 -> IMAPve_g_EMS_MaxTWhl_1/1
  IMAPve_g_EMS_MaxTWhl_Offset/1 -> IMAPve_g_EMS_MaxTWhl_Offset_convert/1
  IMAPve_g_EMS_MaxTWhl_Offset_convert/1 -> IMAPve_g_EMS_MaxTWhl_Offset_1/1
  IMAPve_g_EMS_MinTWhl/1 -> IMAPve_g_EMS_MinTWhl_convert/1
  IMAPve_g_EMS_MinTWhl_convert/1 -> IMAPve_g_EMS_MinTWhl_1/1
  IMAPve_g_EMS_MinTWhl_Offset/1 -> IMAPve_g_EMS_MinTWhl_Offset_convert/1
  IMAPve_g_EMS_MinTWhl_Offset_convert/1 -> IMAPve_g_EMS_MinTWhl_Offset_1/1
  IMAPve_g_EMS_Actual_FlwT/1 -> IMAPve_g_EMS_Actual_FlwT_convert/1
  IMAPve_g_EMS_Actual_FlwT_convert/1 -> IMAPve_g_EMS_Actual_FlwT_1/1
  IMAPve_g_EMS_Actual_IndT/1 -> IMAPve_g_EMS_Actual_IndT_convert/1
  IMAPve_g_EMS_Actual_IndT_convert/1 -> IMAPve_g_EMS_Actual_IndT_1/1
  IMAPve_g_EMS_Realize_TWhl/1 -> IMAPve_g_EMS_Realize_TWhl_convert/1
  IMAPve_g_EMS_Realize_TWhl_convert/1 -> IMAPve_g_EMS_Realize_TWhl_1/1
  IMAPve_g_EMS_ACC_VirtualPedal/1 -> IMAPve_g_EMS_ACC_VirtualPedal_convert/1
  IMAPve_g_EMS_ACC_VirtualPedal_convert/1 -> IMAPve_g_EMS_ACC_VirtualPedal_1/1
  IMAPve_d_EMS_AccPedal_Fault/1 -> IMAPve_d_EMS_AccPedal_Fault_convert/1
  IMAPve_d_EMS_AccPedal_Fault_convert/1 -> IMAPve_d_EMS_AccPedal_Fault_1/1
  IMAPve_g_EMS_Driver_Torque/1 -> IMAPve_g_EMS_Driver_Torque_convert/1
  IMAPve_g_EMS_Driver_Torque_convert/1 -> IMAPve_g_EMS_Driver_Torque_1/1
  IMAPve_d_ESC_Brake_Effort/1 -> IMAPve_d_ESC_Brake_Effort_convert/1
  IMAPve_d_ESC_Brake_Effort_convert/1 -> IMAPve_d_ESC_Brake_Effort_1/1
  IMAPve_g_EMS_Engine_Speed/1 -> IMAPve_g_EMS_Engine_Speed_convert/1
  IMAPve_g_EMS_Engine_Speed_convert/1 -> IMAPve_g_EMS_Engine_Speed_1/1
  IMAPve_d_ESC_Veh_Standstill/1 -> IMAPve_d_ESC_Veh_Standstill_convert/1
  IMAPve_d_ESC_Veh_Standstill_convert/1 -> IMAPve_d_ESC_Veh_Standstill_1/1
  IMAPve_d_TCU_Actual_Gear/1 -> IMAPve_d_TCU_Actual_Gear_convert/1
  IMAPve_d_TCU_Actual_Gear_convert/1 -> IMAPve_d_TCU_Actual_Gear_1/1
  IMAPve_d_TCU_Target_Gear/1 -> IMAPve_d_TCU_Target_Gear_convert/1
  IMAPve_d_TCU_Target_Gear_convert/1 -> IMAPve_d_TCU_Target_Gear_1/1
  IMAPve_d_TCU_PRND_State/1 -> IMAPve_d_TCU_PRND_State_convert/1
  IMAPve_d_TCU_PRND_State_convert/1 -> IMAPve_d_TCU_PRND_State_1/1
  IMAPve_d_BCM_Ignition_State/1 -> IMAPve_d_BCM_Ignition_State_convert/1
  IMAPve_d_BCM_Ignition_State_convert/1 -> IMAPve_d_BCM_Ignition_State_1/1
  IMAPve_d_ACU_Driver_Belt/1 -> IMAPve_d_ACU_Driver_Belt_convert/1
  IMAPve_d_ACU_Driver_Belt_convert/1 -> IMAPve_d_ACU_Driver_Belt_1/1
  IMAPve_d_SWS_Fault_Code/1 -> IMAPve_d_SWS_Fault_Code_convert/1
  IMAPve_d_SWS_Fault_Code_convert/1 -> IMAPve_d_SWS_Fault_Code_1/1
  IMAPve_d_SWS_Failure_Status/1 -> IMAPve_d_SWS_Failure_Status_convert/1
  IMAPve_d_SWS_Failure_Status_convert/1 -> IMAPve_d_SWS_Failure_Status_1/1
  IMAPve_d_ESC_OFF/1 -> IMAPve_d_ESC_OFF_convert/1
  IMAPve_d_ESC_OFF_convert/1 -> IMAPve_d_ESC_OFF_1/1
  IMAPve_d_ESC_AlarmSig/1 -> IMAPve_d_ESC_AlarmSig_convert/1
  IMAPve_d_ESC_AlarmSig_convert/1 -> IMAPve_d_ESC_AlarmSig_1/1
  IMAPve_d_Speed_Limit_Switch/1 -> IMAPve_d_Speed_Limit_Switch_convert/1
  IMAPve_d_Speed_Limit_Switch_convert/1 -> IMAPve_d_Speed_Limit_Switch_1/1
  IMAPve_d_ESC_ESC_Active/1 -> IMAPve_d_ESC_ESC_Active_convert/1
  IMAPve_d_ESC_ESC_Active_convert/1 -> IMAPve_d_ESC_ESC_Active_1/1
  IMAPve_d_ESC_MSR_Active/1 -> IMAPve_d_ESC_MSR_Active_convert/1
  IMAPve_d_ESC_MSR_Active_convert/1 -> IMAPve_d_ESC_MSR_Active_1/1
  IMAPve_d_ESC_TCS_Active/1 -> IMAPve_d_ESC_TCS_Active_convert/1
  IMAPve_d_ESC_TCS_Active_convert/1 -> IMAPve_d_ESC_TCS_Active_1/1
  IMAPve_d_ESC_VehSpd_Valid/1 -> IMAPve_d_ESC_VehSpd_Valid_convert/1
  IMAPve_d_ESC_VehSpd_Valid_convert/1 -> IMAPve_d_ESC_VehSpd_Valid_1/1
  IMAPve_d_Brake_Pedal_Fault/1 -> IMAPve_d_Brake_Pedal_Fault_convert/1
  IMAPve_d_Brake_Pedal_Fault_convert/1 -> IMAPve_d_Brake_Pedal_Fault_1/1
  IMAPve_d_ESC_ABS_Active/1 -> IMAPve_d_ESC_ABS_Active_convert/1
  IMAPve_d_ESC_ABS_Active_convert/1 -> IMAPve_d_ESC_ABS_Active_1/1
  IMAPve_d_ESC_ABS_Valid/1 -> IMAPve_d_ESC_ABS_Valid_convert/1
  IMAPve_d_ESC_ABS_Valid_convert/1 -> IMAPve_d_ESC_ABS_Valid_1/1
  IMAPve_d_ESC_ABS_AlarmSig/1 -> IMAPve_d_ESC_ABS_AlarmSig_convert/1
  IMAPve_d_ESC_ABS_AlarmSig_convert/1 -> IMAPve_d_ESC_ABS_AlarmSig_1/1
  IMAPve_d_ESC_FL_WheelPulVal/1 -> IMAPve_d_ESC_FL_WheelPulVal_convert/1
  IMAPve_d_ESC_FL_WheelPulVal_convert/1 -> IMAPve_d_ESC_FL_WheelPulVal_1/1
  IMAPve_d_ESC_FR_WheelPulVal/1 -> IMAPve_d_ESC_FR_WheelPulVal_convert/1
  IMAPve_d_ESC_FR_WheelPulVal_convert/1 -> IMAPve_d_ESC_FR_WheelPulVal_1/1
  IMAPve_d_ESC_RL_WheelPulVal/1 -> IMAPve_d_ESC_RL_WheelPulVal_convert/1
  IMAPve_d_ESC_RL_WheelPulVal_convert/1 -> IMAPve_d_ESC_RL_WheelPulVal_1/1
  IMAPve_d_ESC_RR_WheelPulVal/1 -> IMAPve_d_ESC_RR_WheelPulVal_convert/1
  IMAPve_d_ESC_RR_WheelPulVal_convert/1 -> IMAPve_d_ESC_RR_WheelPulVal_1/1
  IMAPve_g_ESC_FL_WhlSpd/1 -> IMAPve_g_ESC_FL_WhlSpd_convert/1
  IMAPve_g_ESC_FL_WhlSpd_convert/1 -> IMAPve_g_ESC_FL_WhlSpd_1/1
  IMAPve_d_ESC_FL_WhlSpd_Fault/1 -> IMAPve_d_ESC_FL_WhlSpd_Fault_convert/1
  IMAPve_d_ESC_FL_WhlSpd_Fault_convert/1 -> IMAPve_d_ESC_FL_WhlSpd_Fault_1/1
  IMAPve_g_ESC_FR_WhlSpd/1 -> IMAPve_g_ESC_FR_WhlSpd_convert/1
  IMAPve_g_ESC_FR_WhlSpd_convert/1 -> IMAPve_g_ESC_FR_WhlSpd_1/1
  IMAPve_d_ESC_FR_WhlSpd_Fault/1 -> IMAPve_d_ESC_FR_WhlSpd_Fault_convert/1
  IMAPve_d_ESC_FR_WhlSpd_Fault_convert/1 -> IMAPve_d_ESC_FR_WhlSpd_Fault_1/1
  IMAPve_g_ESC_RL_WhlSpd/1 -> IMAPve_g_ESC_RL_WhlSpd_convert/1
  IMAPve_g_ESC_RL_WhlSpd_convert/1 -> IMAPve_g_ESC_RL_WhlSpd_1/1
  IMAPve_d_ESC_RL_WhlSpd_Fault/1 -> IMAPve_d_ESC_RL_WhlSpd_Fault_convert/1
  IMAPve_d_ESC_RL_WhlSpd_Fault_convert/1 -> IMAPve_d_ESC_RL_WhlSpd_Fault_1/1
  IMAPve_g_ESC_RR_WhlSpd/1 -> IMAPve_g_ESC_RR_WhlSpd_convert/1
  IMAPve_g_ESC_RR_WhlSpd_convert/1 -> IMAPve_g_ESC_RR_WhlSpd_1/1
  IMAPve_d_ESC_RR_WhlSpd_Fault/1 -> IMAPve_d_ESC_RR_WhlSpd_Fault_convert/1
  IMAPve_d_ESC_RR_WhlSpd_Fault_convert/1 -> IMAPve_d_ESC_RR_WhlSpd_Fault_1/1
  IMAPve_d_ESC_FL_Wheel_Pulse/1 -> IMAPve_d_ESC_FL_Wheel_Pulse_convert/1
  IMAPve_d_ESC_FL_Wheel_Pulse_convert/1 -> IMAPve_d_ESC_FL_Wheel_Pulse_1/1
  IMAPve_d_ESC_FR_Wheel_Pulse/1 -> IMAPve_d_ESC_FR_Wheel_Pulse_convert/1
  IMAPve_d_ESC_FR_Wheel_Pulse_convert/1 -> IMAPve_d_ESC_FR_Wheel_Pulse_1/1
  IMAPve_d_ESC_RL_Wheel_Pulse/1 -> IMAPve_d_ESC_RL_Wheel_Pulse_convert/1
  IMAPve_d_ESC_RL_Wheel_Pulse_convert/1 -> IMAPve_d_ESC_RL_Wheel_Pulse_1/1
  IMAPve_d_ESC_RR_Wheel_Pulse/1 -> IMAPve_d_ESC_RR_Wheel_Pulse_convert/1
  IMAPve_d_ESC_RR_Wheel_Pulse_convert/1 -> IMAPve_d_ESC_RR_Wheel_Pulse_1/1
  IMAPve_d_TCU_AT_Failure/1 -> IMAPve_d_TCU_AT_Failure_convert/1
  IMAPve_d_TCU_AT_Failure_convert/1 -> IMAPve_d_TCU_AT_Failure_1/1
  IMAPve_d_TCU_Shift_Valid/1 -> IMAPve_d_TCU_Shift_Valid_convert/1
  IMAPve_d_TCU_Shift_Valid_convert/1 -> IMAPve_d_TCU_Shift_Valid_1/1
  IMAPve_d_TCU_DCT_Clutch_State/1 -> IMAPve_d_TCU_DCT_Clutch_State_convert/1
  IMAPve_d_TCU_DCT_Clutch_State_convert/1 -> IMAPve_d_TCU_DCT_Clutch_State_1/1
  IMAPve_d_TCU_Gear_Engage/1 -> IMAPve_d_TCU_Gear_Engage_convert/1
  IMAPve_d_TCU_Gear_Engage_convert/1 -> IMAPve_d_TCU_Gear_Engage_1/1
  IMAPve_d_TCU_Select_ATMode/1 -> IMAPve_d_TCU_Select_ATMode_convert/1
  IMAPve_d_TCU_Select_ATMode_convert/1 -> IMAPve_d_TCU_Select_ATMode_1/1
  IMAPve_d_EMS_Engine_Status/1 -> IMAPve_d_EMS_Engine_Status_convert/1
  IMAPve_d_EMS_Engine_Status_convert/1 -> IMAPve_d_EMS_Engine_Status_1/1
  IMAPve_d_EMS_Gearbox_CtlAvail/1 -> IMAPve_d_EMS_Gearbox_CtlAvail_convert/1
  IMAPve_d_EMS_Gearbox_CtlAvail_convert/1 -> IMAPve_d_EMS_Gearbox_CtlAvail_1/1
  IMAPve_d_ESC_Brake_Failsafe/1 -> IMAPve_d_ESC_Brake_Failsafe_convert/1
  IMAPve_d_ESC_Brake_Failsafe_convert/1 -> IMAPve_d_ESC_Brake_Failsafe_1/1
  IMAPve_d_ESC_AEB_Status/1 -> IMAPve_d_ESC_AEB_Status_convert/1
  IMAPve_d_ESC_AEB_Status_convert/1 -> IMAPve_d_ESC_AEB_Status_1/1
  IMAPve_d_ESC_AEB_Available/1 -> IMAPve_d_ESC_AEB_Available_convert/1
  IMAPve_d_ESC_AEB_Available_convert/1 -> IMAPve_d_ESC_AEB_Available_1/1
  IMAPve_d_ESC_AEB_Active/1 -> IMAPve_d_ESC_AEB_Active_convert/1
  IMAPve_d_ESC_AEB_Active_convert/1 -> IMAPve_d_ESC_AEB_Active_1/1
  IMAPve_d_ESC_ACC_Status/1 -> IMAPve_d_ESC_ACC_Status_convert/1
  IMAPve_d_ESC_ACC_Status_convert/1 -> IMAPve_d_ESC_ACC_Status_1/1
  IMAPve_d_ESC_ACC_Available/1 -> IMAPve_d_ESC_ACC_Available_convert/1
  IMAPve_d_ESC_ACC_Available_convert/1 -> IMAPve_d_ESC_ACC_Available_1/1
  IMAPve_d_ESC_ACC_Active/1 -> IMAPve_d_ESC_ACC_Active_convert/1
  IMAPve_d_ESC_ACC_Active_convert/1 -> IMAPve_d_ESC_ACC_Active_1/1
  IMAPve_d_EMS_ACC_Effective/1 -> IMAPve_d_EMS_ACC_Effective_convert/1
  IMAPve_d_EMS_ACC_Effective_convert/1 -> IMAPve_d_EMS_ACC_Effective_1/1
  IMAPve_d_BCM_FrontWiper_State/1 -> IMAPve_d_BCM_FrontWiper_State_convert/1
  IMAPve_d_BCM_FrontWiper_State_convert/1 -> IMAPve_d_BCM_FrontWiper_State_1/1
  IMAPve_d_BCM_CHMSL_Status/1 -> IMAPve_d_BCM_CHMSL_Status_convert/1
  IMAPve_d_BCM_CHMSL_Status_convert/1 -> IMAPve_d_BCM_CHMSL_Status_1/1
  IMAPve_d_BCM_BrakeLamp_State/1 -> IMAPve_d_BCM_BrakeLamp_State_convert/1
  IMAPve_d_BCM_BrakeLamp_State_convert/1 -> IMAPve_d_BCM_BrakeLamp_State_1/1
  IMAPve_d_GW_Brake_Only_Req/1 -> IMAPve_d_GW_Brake_Only_Req_convert/1
  IMAPve_d_GW_Brake_Only_Req_convert/1 -> IMAPve_d_GW_Brake_Only_Req_1/1
  IMAPve_d_ACU_Passenger_Belt/1 -> IMAPve_d_ACU_Passenger_Belt_convert/1
  IMAPve_d_ACU_Passenger_Belt_convert/1 -> IMAPve_d_ACU_Passenger_Belt_1/1
  IMAPve_d_EMS_ACC_CtlAvail/1 -> IMAPve_d_EMS_ACC_CtlAvail_convert/1
  IMAPve_d_EMS_ACC_CtlAvail_convert/1 -> IMAPve_d_EMS_ACC_CtlAvail_1/1
  IMAPve_d_EMS_ACC_Inhibited/1 -> IMAPve_d_EMS_ACC_Inhibited_convert/1
  IMAPve_d_EMS_ACC_Inhibited_convert/1 -> IMAPve_d_EMS_ACC_Inhibited_1/1
  IMAPve_d_EMS_Brake_Pedal/1 -> IMAPve_d_EMS_Brake_Pedal_convert/1
  IMAPve_d_EMS_Brake_Pedal_convert/1 -> IMAPve_d_EMS_Brake_Pedal_1/1
  IMAPve_d_BCM_LowBeam_State/1 -> IMAPve_d_BCM_LowBeam_State_convert/1
  IMAPve_d_BCM_LowBeam_State_convert/1 -> IMAPve_d_BCM_LowBeam_State_1/1
  IMAPve_d_BCM_HighBeam_State/1 -> IMAPve_d_BCM_HighBeam_State_convert/1
  IMAPve_d_BCM_HighBeam_State_convert/1 -> IMAPve_d_BCM_HighBeam_State_1/1
  IMAPve_d_EPB_Status/1 -> IMAPve_d_EPB_Status_convert/1
  IMAPve_d_EPB_Status_convert/1 -> IMAPve_d_EPB_Status_1/1
  IMAPve_d_EPB_Display_Req/1 -> IMAPve_d_EPB_Display_Req_convert/1
  IMAPve_d_EPB_Display_Req_convert/1 -> IMAPve_d_EPB_Display_Req_1/1
  IMAPve_d_EPB_Warn_Req/1 -> IMAPve_d_EPB_Warn_Req_convert/1
  IMAPve_d_EPB_Warn_Req_convert/1 -> IMAPve_d_EPB_Warn_Req_1/1
  IMAPve_d_EPB_Switch_State/1 -> IMAPve_d_EPB_Switch_State_convert/1
  IMAPve_d_EPB_Switch_State_convert/1 -> IMAPve_d_EPB_Switch_State_1/1
  IMAPve_d_EPB_Switch_Valid/1 -> IMAPve_d_EPB_Switch_Valid_convert/1
  IMAPve_d_EPB_Switch_Valid_convert/1 -> IMAPve_d_EPB_Switch_Valid_1/1
  IMAPve_d_ESC_Drive_Direction/1 -> IMAPve_d_ESC_Drive_Direction_convert/1
  IMAPve_d_ESC_Drive_Direction_convert/1 -> IMAPve_d_ESC_Drive_Direction_1/1
  IMAPve_d_ESC_Hold_State/1 -> IMAPve_d_ESC_Hold_State_convert/1
  IMAPve_d_ESC_Hold_State_convert/1 -> IMAPve_d_ESC_Hold_State_1/1
  IMAPve_d_EPS_Steer_Hold_State/1 -> IMAPve_d_EPS_Steer_Hold_State_convert/1
  IMAPve_d_EPS_Steer_Hold_State_convert/1 -> IMAPve_d_EPS_Steer_Hold_State_1/1
  IMAPve_d_EPS_Warning_State/1 -> IMAPve_d_EPS_Warning_State_convert/1
  IMAPve_d_EPS_Warning_State_convert/1 -> IMAPve_d_EPS_Warning_State_1/1
  IMAPve_g_EPS_PowerCon/1 -> IMAPve_g_EPS_PowerCon_convert/1
  IMAPve_g_EPS_PowerCon_convert/1 -> IMAPve_g_EPS_PowerCon_1/1
  IMAPve_d_ESC_EBD_AlarmSig/1 -> IMAPve_d_ESC_EBD_AlarmSig_convert/1
  IMAPve_d_ESC_EBD_AlarmSig_convert/1 -> IMAPve_d_ESC_EBD_AlarmSig_1/1
  IMAPve_d_ESC_AVH_Status/1 -> IMAPve_d_ESC_AVH_Status_convert/1
  IMAPve_d_ESC_AVH_Status_convert/1 -> IMAPve_d_ESC_AVH_Status_1/1
  IMAPve_d_Radar_Detective_Req/1 -> IMAPve_d_Radar_Detective_Req_convert/1
  IMAPve_d_Radar_Detective_Req_convert/1 -> IMAPve_d_Radar_Detective_Req_1/1
  IMAPve_g_BCM_Battery_Voltage/1 -> IMAPve_g_BCM_Battery_Voltage_convert/1
  IMAPve_g_BCM_Battery_Voltage_convert/1 -> IMAPve_g_BCM_Battery_Voltage_1/1
  IMAPve_d_TBOX_LocalTimeY/1 -> IMAPve_d_TBOX_LocalTimeY_convert/1
  IMAPve_d_TBOX_LocalTimeY_convert/1 -> IMAPve_d_TBOX_LocalTimeY_1/1
  IMAPve_d_TBOX_LocalTimeM/1 -> IMAPve_d_TBOX_LocalTimeM_convert/1
  IMAPve_d_TBOX_LocalTimeM_convert/1 -> IMAPve_d_TBOX_LocalTimeM_1/1
  IMAPve_d_TBOX_LocalTimeD/1 -> IMAPve_d_TBOX_LocalTimeD_convert/1
  IMAPve_d_TBOX_LocalTimeD_convert/1 -> IMAPve_d_TBOX_LocalTimeD_1/1
  IMAPve_d_TBOX_LocalTimeH/1 -> IMAPve_d_TBOX_LocalTimeH_convert/1
  IMAPve_d_TBOX_LocalTimeH_convert/1 -> IMAPve_d_TBOX_LocalTimeH_1/1
  IMAPve_d_TBOX_LocalTimeMin/1 -> IMAPve_d_TBOX_LocalTimeMin_convert/1
  IMAPve_d_TBOX_LocalTimeMin_convert/1 -> IMAPve_d_TBOX_LocalTimeMin_1/1
  IMAPve_d_TBOX_LocalTimeS/1 -> IMAPve_d_TBOX_LocalTimeS_convert/1
  IMAPve_d_TBOX_LocalTimeS_convert/1 -> IMAPve_d_TBOX_LocalTimeS_1/1
  IMAPve_d_TBOX_LocalTime_Valid/1 -> IMAPve_d_TBOX_LocalTime_Valid_convert/1
  IMAPve_d_TBOX_LocalTime_Valid_convert/1 -> IMAPve_d_TBOX_LocalTime_Valid_1/1
  IMAPve_d_TPMS_Warn_Indicate/1 -> IMAPve_d_TPMS_Warn_Indicate_convert/1
  IMAPve_d_TPMS_Warn_Indicate_convert/1 -> IMAPve_d_TPMS_Warn_Indicate_1/1
  IMAPve_d_Radar_State/1 -> IMAPve_d_Radar_State_convert/1
  IMAPve_d_Radar_State_convert/1 -> IMAPve_d_Radar_State_1/1
  IMAPve_d_ACC_Desired_Headway/1 -> IMAPve_d_ACC_Desired_Headway_convert/1
  IMAPve_d_ACC_Desired_Headway_convert/1 -> IMAPve_d_ACC_Desired_Headway_1/1
  IMAPve_d_Time_System_Clock/1 -> IMAPve_d_Time_System_Clock_convert/1
  IMAPve_d_Time_System_Clock_convert/1 -> IMAPve_d_Time_System_Clock_1/1
  IMAPve_d_Signal_Time_Stamp/1 -> IMAPve_d_Signal_Time_Stamp_convert/1
  IMAPve_d_Signal_Time_Stamp_convert/1 -> IMAPve_d_Signal_Time_Stamp_1/1
  IMAPve_g_GW_IC_Odometer/1 -> IMAPve_g_GW_IC_Odometer_convert/1
  IMAPve_g_GW_IC_Odometer_convert/1 -> IMAPve_g_GW_IC_Odometer_1/1
  IMAPve_g_FAPA_State/1 -> IMAPve_g_FAPA_State_convert/1
  IMAPve_g_FAPA_State_convert/1 -> IMAPve_g_FAPA_State_1/1
  IMAPve_d_Outside_Temp/1 -> IMAPve_d_Outside_Temp_convert/1
  IMAPve_d_Outside_Temp_convert/1 -> IMAPve_d_Outside_Temp_1/1
  IMAPve_d_ORI_CIPV_ID/1 -> IMAPve_d_ORI_CIPV_ID_convert/1
  IMAPve_d_ORI_CIPV_ID_convert/1 -> IMAPve_d_ORI_CIPV_ID_1/1
  IMAPve_d_ORI_Obj_Num/1 -> IMAPve_d_ORI_Obj_Num_convert/1
  IMAPve_d_ORI_Obj_Num_convert/1 -> IMAPve_d_ORI_Obj_Num_1/1
  IMAPva_g_ORI_Probability/1 -> IMAPva_g_ORI_Probability_convert/1
  IMAPva_g_ORI_Probability_convert/1 -> IMAPva_g_ORI_Probability_1/1
  IMAPva_d_ORI_Obj_Class/1 -> IMAPva_d_ORI_Obj_Class_convert/1
  IMAPva_d_ORI_Obj_Class_convert/1 -> IMAPva_d_ORI_Obj_Class_1/1
  IMAPva_d_ORI_Obj_Motion/1 -> IMAPva_d_ORI_Obj_Motion_convert/1
  IMAPva_d_ORI_Obj_Motion_convert/1 -> IMAPva_d_ORI_Obj_Motion_1/1
  IMAPva_g_ORI_Obj_RelVel/1 -> IMAPva_g_ORI_Obj_RelVel_convert/1
  IMAPva_g_ORI_Obj_RelVel_convert/1 -> IMAPva_g_ORI_Obj_RelVel_1/1
  IMAPva_g_ORI_Obj_LongDis/1 -> IMAPva_g_ORI_Obj_LongDis_convert/1
  IMAPva_g_ORI_Obj_LongDis_convert/1 -> IMAPva_g_ORI_Obj_LongDis_1/1
  IMAPva_d_ORI_Obj_Lane/1 -> IMAPva_d_ORI_Obj_Lane_convert/1
  IMAPva_d_ORI_Obj_Lane_convert/1 -> IMAPva_d_ORI_Obj_Lane_1/1
  IMAPva_g_ORI_Obj_LAngle/1 -> IMAPva_g_ORI_Obj_LAngle_convert/1
  IMAPva_g_ORI_Obj_LAngle_convert/1 -> IMAPva_g_ORI_Obj_LAngle_1/1
  IMAPva_g_ORI_Obj_RAngle/1 -> IMAPva_g_ORI_Obj_RAngle_convert/1
  IMAPva_g_ORI_Obj_RAngle_convert/1 -> IMAPva_g_ORI_Obj_RAngle_1/1
  IMAPva_g_ORI_Obj_Width/1 -> IMAPva_g_ORI_Obj_Width_convert/1
  IMAPva_g_ORI_Obj_Width_convert/1 -> IMAPva_g_ORI_Obj_Width_1/1
  IMAPva_d_ORI_Obj_ID/1 -> IMAPva_d_ORI_Obj_ID_convert/1
  IMAPva_d_ORI_Obj_ID_convert/1 -> IMAPva_d_ORI_Obj_ID_1/1
  IMAPve_d_ORI_Lane_Valid/1 -> IMAPve_d_ORI_Lane_Valid_convert/1
  IMAPve_d_ORI_Lane_Valid_convert/1 -> IMAPve_d_ORI_Lane_Valid_1/1
  IMAPve_d_ORI_Lane_ConsArea/1 -> IMAPve_d_ORI_Lane_ConsArea_convert/1
  IMAPve_d_ORI_Lane_ConsArea_convert/1 -> IMAPve_d_ORI_Lane_ConsArea_1/1
  IMAPve_d_ORI_Lane_RoadType/1 -> IMAPve_d_ORI_Lane_RoadType_convert/1
  IMAPve_d_ORI_Lane_RoadType_convert/1 -> IMAPve_d_ORI_Lane_RoadType_1/1
  IMAPve_g_ORI_L0_C3/1 -> IMAPve_g_ORI_L0_C3_convert/1
  IMAPve_g_ORI_L0_C3_convert/1 -> IMAPve_g_ORI_L0_C3_1/1
  IMAPve_g_ORI_L0_C2/1 -> IMAPve_g_ORI_L0_C2_convert/1
  IMAPve_g_ORI_L0_C2_convert/1 -> IMAPve_g_ORI_L0_C2_1/1
  IMAPve_g_ORI_L0_C1/1 -> IMAPve_g_ORI_L0_C1_convert/1
  IMAPve_g_ORI_L0_C1_convert/1 -> IMAPve_g_ORI_L0_C1_1/1
  IMAPve_g_ORI_L0_C0/1 -> IMAPve_g_ORI_L0_C0_convert/1
  IMAPve_g_ORI_L0_C0_convert/1 -> IMAPve_g_ORI_L0_C0_1/1
  IMAPve_d_ORI_L0_Q/1 -> IMAPve_d_ORI_L0_Q_convert/1
  IMAPve_d_ORI_L0_Q_convert/1 -> IMAPve_d_ORI_L0_Q_1/1
  IMAPve_d_ORI_L0_Type/1 -> IMAPve_d_ORI_L0_Type_convert/1
  IMAPve_d_ORI_L0_Type_convert/1 -> IMAPve_d_ORI_L0_Type_1/1
  IMAPve_g_ORI_L0_VR/1 -> IMAPve_g_ORI_L0_VR_convert/1
  IMAPve_g_ORI_L0_VR_convert/1 -> IMAPve_g_ORI_L0_VR_1/1
  IMAPve_g_ORI_L0_TLC/1 -> IMAPve_g_ORI_L0_TLC_convert/1
  IMAPve_g_ORI_L0_TLC_convert/1 -> IMAPve_g_ORI_L0_TLC_1/1
  IMAPve_g_ORI_L0_W/1 -> IMAPve_g_ORI_L0_W_convert/1
  IMAPve_g_ORI_L0_W_convert/1 -> IMAPve_g_ORI_L0_W_1/1
  IMAPve_d_ORI_L0_LC/1 -> IMAPve_d_ORI_L0_LC_convert/1
  IMAPve_d_ORI_L0_LC_convert/1 -> IMAPve_d_ORI_L0_LC_1/1
  IMAPve_g_ORI_L1_C3/1 -> IMAPve_g_ORI_L1_C3_convert/1
  IMAPve_g_ORI_L1_C3_convert/1 -> IMAPve_g_ORI_L1_C3_1/1
  IMAPve_g_ORI_L1_C2/1 -> IMAPve_g_ORI_L1_C2_convert/1
  IMAPve_g_ORI_L1_C2_convert/1 -> IMAPve_g_ORI_L1_C2_1/1
  IMAPve_g_ORI_L1_C1/1 -> IMAPve_g_ORI_L1_C1_convert/1
  IMAPve_g_ORI_L1_C1_convert/1 -> IMAPve_g_ORI_L1_C1_1/1
  IMAPve_g_ORI_L1_C0/1 -> IMAPve_g_ORI_L1_C0_convert/1
  IMAPve_g_ORI_L1_C0_convert/1 -> IMAPve_g_ORI_L1_C0_1/1
  IMAPve_d_ORI_L1_Q/1 -> IMAPve_d_ORI_L1_Q_convert/1
  IMAPve_d_ORI_L1_Q_convert/1 -> IMAPve_d_ORI_L1_Q_1/1
  IMAPve_d_ORI_L1_Type/1 -> IMAPve_d_ORI_L1_Type_convert/1
  IMAPve_d_ORI_L1_Type_convert/1 -> IMAPve_d_ORI_L1_Type_1/1
  IMAPve_g_ORI_L1_VR/1 -> IMAPve_g_ORI_L1_VR_convert/1
  IMAPve_g_ORI_L1_VR_convert/1 -> IMAPve_g_ORI_L1_VR_1/1
  IMAPve_g_ORI_L1_TLC/1 -> IMAPve_g_ORI_L1_TLC_convert/1
  IMAPve_g_ORI_L1_TLC_convert/1 -> IMAPve_g_ORI_L1_TLC_1/1
  IMAPve_g_ORI_L1_W/1 -> IMAPve_g_ORI_L1_W_convert/1
  IMAPve_g_ORI_L1_W_convert/1 -> IMAPve_g_ORI_L1_W_1/1
  IMAPve_d_ORI_L1_LC/1 -> IMAPve_d_ORI_L1_LC_convert/1
  IMAPve_d_ORI_L1_LC_convert/1 -> IMAPve_d_ORI_L1_LC_1/1
  IMAPve_g_ORI_R0_C3/1 -> IMAPve_g_ORI_R0_C3_convert/1
  IMAPve_g_ORI_R0_C3_convert/1 -> IMAPve_g_ORI_R0_C3_1/1
  IMAPve_g_ORI_R0_C2/1 -> IMAPve_g_ORI_R0_C2_convert/1
  IMAPve_g_ORI_R0_C2_convert/1 -> IMAPve_g_ORI_R0_C2_1/1
  IMAPve_g_ORI_R0_C1/1 -> IMAPve_g_ORI_R0_C1_convert/1
  IMAPve_g_ORI_R0_C1_convert/1 -> IMAPve_g_ORI_R0_C1_1/1
  IMAPve_g_ORI_R0_C0/1 -> IMAPve_g_ORI_R0_C0_convert/1
  IMAPve_g_ORI_R0_C0_convert/1 -> IMAPve_g_ORI_R0_C0_1/1
  IMAPve_d_ORI_R0_Q/1 -> IMAPve_d_ORI_R0_Q_convert/1
  IMAPve_d_ORI_R0_Q_convert/1 -> IMAPve_d_ORI_R0_Q_1/1
  IMAPve_d_ORI_R0_LT/1 -> IMAPve_d_ORI_R0_LT_convert/1
  IMAPve_d_ORI_R0_LT_convert/1 -> IMAPve_d_ORI_R0_LT_1/1
  IMAPve_g_ORI_R0_VR/1 -> IMAPve_g_ORI_R0_VR_convert/1
  IMAPve_g_ORI_R0_VR_convert/1 -> IMAPve_g_ORI_R0_VR_1/1
  IMAPve_g_ORI_R0_TLC/1 -> IMAPve_g_ORI_R0_TLC_convert/1
  IMAPve_g_ORI_R0_TLC_convert/1 -> IMAPve_g_ORI_R0_TLC_1/1
  IMAPve_g_ORI_R0_W/1 -> IMAPve_g_ORI_R0_W_convert/1
  IMAPve_g_ORI_R0_W_convert/1 -> IMAPve_g_ORI_R0_W_1/1
  IMAPve_d_ORI_R0_LC/1 -> IMAPve_d_ORI_R0_LC_convert/1
  IMAPve_d_ORI_R0_LC_convert/1 -> IMAPve_d_ORI_R0_LC_1/1
  IMAPve_g_ORI_R1_C3/1 -> IMAPve_g_ORI_R1_C3_convert/1
  IMAPve_g_ORI_R1_C3_convert/1 -> IMAPve_g_ORI_R1_C3_1/1
  IMAPve_g_ORI_R1_C2/1 -> IMAPve_g_ORI_R1_C2_convert/1
  IMAPve_g_ORI_R1_C2_convert/1 -> IMAPve_g_ORI_R1_C2_1/1
  IMAPve_g_ORI_R1_C1/1 -> IMAPve_g_ORI_R1_C1_convert/1
  IMAPve_g_ORI_R1_C1_convert/1 -> IMAPve_g_ORI_R1_C1_1/1
  IMAPve_g_ORI_R1_C0/1 -> IMAPve_g_ORI_R1_C0_convert/1
  IMAPve_g_ORI_R1_C0_convert/1 -> IMAPve_g_ORI_R1_C0_1/1
  IMAPve_d_ORI_R1_Q/1 -> IMAPve_d_ORI_R1_Q_convert/1
  IMAPve_d_ORI_R1_Q_convert/1 -> IMAPve_d_ORI_R1_Q_1/1
  IMAPve_d_ORI_R1_LT/1 -> IMAPve_d_ORI_R1_LT_convert/1
  IMAPve_d_ORI_R1_LT_convert/1 -> IMAPve_d_ORI_R1_LT_1/1
  IMAPve_g_ORI_R1_VR/1 -> IMAPve_g_ORI_R1_VR_convert/1
  IMAPve_g_ORI_R1_VR_convert/1 -> IMAPve_g_ORI_R1_VR_1/1
  IMAPve_g_ORI_R1_TLC/1 -> IMAPve_g_ORI_R1_TLC_convert/1
  IMAPve_g_ORI_R1_TLC_convert/1 -> IMAPve_g_ORI_R1_TLC_1/1
  IMAPve_g_ORI_R1_W/1 -> IMAPve_g_ORI_R1_W_convert/1
  IMAPve_g_ORI_R1_W_convert/1 -> IMAPve_g_ORI_R1_W_1/1
  IMAPve_d_ORI_R1_LC/1 -> IMAPve_d_ORI_R1_LC_convert/1
  IMAPve_d_ORI_R1_LC_convert/1 -> IMAPve_d_ORI_R1_LC_1/1
  IMAPve_d_Sensor_Status/1 -> IMAPve_d_Sensor_Status_convert/1
  IMAPve_d_Sensor_Status_convert/1 -> IMAPve_d_Sensor_Status_1/1
  IMAPve_d_LF_Radar_Status/1 -> IMAPve_d_LF_Radar_Status_convert/1
  IMAPve_d_LF_Radar_Status_convert/1 -> IMAPve_d_LF_Radar_Status_1/1
  IMAPve_d_RF_Radar_Status/1 -> IMAPve_d_RF_Radar_Status_convert/1
  IMAPve_d_RF_Radar_Status_convert/1 -> IMAPve_d_RF_Radar_Status_1/1
  IMAPve_d_LR_Radar_Status/1 -> IMAPve_d_LR_Radar_Status_convert/1
  IMAPve_d_LR_Radar_Status_convert/1 -> IMAPve_d_LR_Radar_Status_1/1
  IMAPve_d_RR_Radar_Status/1 -> IMAPve_d_RR_Radar_Status_convert/1
  IMAPve_d_RR_Radar_Status_convert/1 -> IMAPve_d_RR_Radar_Status_1/1
  IMAPve_d_Fusion_Status/1 -> IMAPve_d_Fusion_Status_convert/1
  IMAPve_d_Fusion_Status_convert/1 -> IMAPve_d_Fusion_Status_1/1
  IMAPve_g_Fusion_Time_Stamp/1 -> IMAPve_g_Fusion_Time_Stamp_convert/1
  IMAPve_g_Fusion_Time_Stamp_convert/1 -> IMAPve_g_Fusion_Time_Stamp_1/1
  IMAPve_d_obj_Num/1 -> IMAPve_d_obj_Num_convert/1
  IMAPve_d_obj_Num_convert/1 -> IMAPve_d_obj_Num_1/1
  IMAPva_d_obj_id_convert/1 -> IMAPva_d_obj_id_1/1
  IMAPva_g_obj_pos_x/1 -> IMAPva_g_obj_pos_x_convert/1  "IMAPva_g_obj_pos_x"
  IMAPva_g_obj_pos_x_convert/1 -> IMAPva_g_obj_pos_x_1/1
  IMAPva_g_obj_pos_y/1 -> IMAPva_g_obj_pos_y_convert/1  "IMAPva_g_obj_pos_y"
  IMAPva_g_obj_pos_y_convert/1 -> IMAPva_g_obj_pos_y_1/1
  IMAPva_g_obj_vel_x/1 -> IMAPva_g_obj_vel_x_convert/1  "IMAPva_g_obj_vel_x"
  IMAPva_g_obj_vel_x_convert/1 -> IMAPva_g_obj_vel_x_1/1
  IMAPva_g_obj_vel_y/1 -> IMAPva_g_obj_vel_y_convert/1  "IMAPva_g_obj_vel_y"
  IMAPva_g_obj_vel_y_convert/1 -> IMAPva_g_obj_vel_y_1/1
  IMAPva_g_obj_acc_x/1 -> IMAPva_g_obj_acc_x_convert/1  "IMAPva_g_obj_acc_x"
  IMAPva_g_obj_acc_x_convert/1 -> IMAPva_g_obj_acc_x_1/1
  IMAPva_g_obj_acc_y/1 -> IMAPva_g_obj_acc_y_convert/1  "IMAPva_g_obj_acc_y"
  IMAPva_g_obj_acc_y_convert/1 -> IMAPva_g_obj_acc_y_1/1
  IMAPva_g_obj_pos_var_x/1 -> IMAPva_g_obj_pos_var_x_convert/1  "IMAPva_g_obj_pos_var_x"
  IMAPva_g_obj_pos_var_x_convert/1 -> IMAPva_g_obj_pos_var_x_1/1
  IMAPva_g_obj_pos_var_y/1 -> IMAPva_g_obj_pos_var_y_convert/1  "IMAPva_g_obj_pos_var_y"
  IMAPva_g_obj_pos_var_y_convert/1 -> IMAPva_g_obj_pos_var_y_1/1
  IMAPva_g_obj_pos_var_xy/1 -> IMAPva_g_obj_pos_var_xy_convert/1  "IMAPva_g_obj_pos_var_xy"
  IMAPva_g_obj_pos_var_xy_convert/1 -> IMAPva_g_obj_pos_var_xy_1/1
  IMAPva_g_obj_vel_var_x/1 -> IMAPva_g_obj_vel_var_x_convert/1  "IMAPva_g_obj_vel_var_x"
  IMAPva_g_obj_vel_var_x_convert/1 -> IMAPva_g_obj_vel_var_x_1/1
  IMAPva_g_obj_vel_var_y/1 -> IMAPva_g_obj_vel_var_y_convert/1  "IMAPva_g_obj_vel_var_y"
  IMAPva_g_obj_vel_var_y_convert/1 -> IMAPva_g_obj_vel_var_y_1/1
  IMAPva_g_obj_vel_var_xy/1 -> IMAPva_g_obj_vel_var_xy_convert/1  "IMAPva_g_obj_vel_var_xy"
  IMAPva_g_obj_vel_var_xy_convert/1 -> IMAPva_g_obj_vel_var_xy_1/1
  IMAPva_g_obj_width/1 -> IMAPva_g_obj_width_convert/1  "IMAPva_g_obj_width"
  IMAPva_g_obj_width_convert/1 -> IMAPva_g_obj_width_1/1
  IMAPva_g_obj_length/1 -> IMAPva_g_obj_length_convert/1  "IMAPva_g_obj_length"
  IMAPva_g_obj_length_convert/1 -> IMAPva_g_obj_length_1/1
  IMAPva_d_obj_fusion_type/1 -> IMAPva_d_obj_fusion_type_convert/1  "IMAPva_d_obj_fusion_type"
  IMAPva_d_obj_fusion_type_convert/1 -> IMAPva_d_obj_fusion_type_1/1
  IMAPva_d_obj_class/1 -> IMAPva_d_obj_class_convert/1  "IMAPva_d_obj_class"
  IMAPva_d_obj_class_convert/1 -> IMAPva_d_obj_class_1/1
  IMAPva_d_obj_lane/1 -> IMAPva_d_obj_lane_convert/1  "IMAPva_d_obj_lane"
  IMAPva_d_obj_lane_convert/1 -> IMAPva_d_obj_lane_1/1
  IMAPva_d_obj_status/1 -> IMAPva_d_obj_status_convert/1  "IMAPva_d_obj_status"
  IMAPva_d_obj_status_convert/1 -> IMAPva_d_obj_status_1/1
  IMAPva_d_obj_cam_asso_id/1 -> IMAPva_d_obj_cam_asso_id_convert/1
  IMAPva_d_obj_cam_asso_id_convert/1 -> IMAPva_d_obj_cam_asso_id_1/1
  IMAPva_g_obj_con_convert/1 -> IMAPva_g_obj_con_1/1
  IMAPva_g_obj_age/1 -> IMAPva_g_obj_age_convert/1  "IMAPva_g_obj_age"
  IMAPva_g_obj_age_convert/1 -> IMAPva_g_obj_age_1/1
  IMAPva_d_obj_TurnLight/1 -> IMAPva_d_obj_TurnLight_convert/1  "IMAPva_d_obj_TurnLight"
  IMAPva_d_obj_TurnLight_convert/1 -> IMAPva_d_obj_TurnLight_1/1
  IMAPva_d_obj_BrakeLight/1 -> IMAPva_d_obj_BrakeLight_convert/1  "IMAPva_d_obj_BrakeLight"
  IMAPva_d_obj_BrakeLight_convert/1 -> IMAPva_d_obj_BrakeLight_1/1
  IMAPva_d_obj_MotionStatus_convert/1 -> IMAPva_d_obj_MotionStatus_1/1
  IMAPva_d_obj_ACC/1 -> IMAPva_d_obj_ACC_convert/1
  IMAPva_d_obj_ACC_convert/1 -> IMAPva_d_obj_ACC_1/1
  IMAPva_d_obj_AEB/1 -> IMAPva_d_obj_AEB_convert/1
  IMAPva_d_obj_AEB_convert/1 -> IMAPva_d_obj_AEB_1/1
  IMAPva_d_obj_ELK/1 -> IMAPva_d_obj_ELK_convert/1
  IMAPva_d_obj_ELK_convert/1 -> IMAPva_d_obj_ELK_1/1
  IMAPva_d_obj_ALC/1 -> IMAPva_d_obj_ALC_convert/1
  IMAPva_d_obj_ALC_convert/1 -> IMAPva_d_obj_ALC_1/1
  IMAPva_d_obj_ESA/1 -> IMAPva_d_obj_ESA_convert/1
  IMAPva_d_obj_ESA_convert/1 -> IMAPva_d_obj_ESA_1/1
  IMAPva_d_obj_JA/1 -> IMAPva_d_obj_JA_convert/1
  IMAPva_d_obj_JA_convert/1 -> IMAPva_d_obj_JA_1/1
  IMAPve_d_Lane_Valid/1 -> IMAPve_d_Lane_Valid_convert/1
  IMAPve_d_Lane_Valid_convert/1 -> IMAPve_d_Lane_Valid_1/1
  IMAPve_d_Road_Type/1 -> IMAPve_d_Road_Type_convert/1
  IMAPve_d_Road_Type_convert/1 -> IMAPve_d_Road_Type_1/1
  IMAPve_d_ConsArea/1 -> IMAPve_d_ConsArea_convert/1
  IMAPve_d_ConsArea_convert/1 -> IMAPve_d_ConsArea_1/1
  IMAPve_g_L0_C0/1 -> IMAPve_g_L0_C0_convert/1
  IMAPve_g_L0_C0_convert/1 -> IMAPve_g_L0_C0_1/1
  IMAPve_g_L0_C1/1 -> IMAPve_g_L0_C1_convert/1
  IMAPve_g_L0_C1_convert/1 -> IMAPve_g_L0_C1_1/1
  IMAPve_g_L0_C2/1 -> IMAPve_g_L0_C2_convert/1
  IMAPve_g_L0_C2_convert/1 -> IMAPve_g_L0_C2_1/1
  IMAPve_g_L0_C3/1 -> IMAPve_g_L0_C3_convert/1
  IMAPve_g_L0_C3_convert/1 -> IMAPve_g_L0_C3_1/1
  IMAPve_g_L0_VR/1 -> IMAPve_g_L0_VR_convert/1
  IMAPve_g_L0_VR_convert/1 -> IMAPve_g_L0_VR_1/1
  IMAPve_d_L0_Q/1 -> IMAPve_d_L0_Q_convert/1
  IMAPve_d_L0_Q_convert/1 -> IMAPve_d_L0_Q_1/1
  IMAPve_d_L0_Type/1 -> IMAPve_d_L0_Type_convert/1
  IMAPve_d_L0_Type_convert/1 -> IMAPve_d_L0_Type_1/1
  IMAPve_g_L0_Confidence/1 -> IMAPve_g_L0_Confidence_convert/1
  IMAPve_g_L0_Confidence_convert/1 -> IMAPve_g_L0_Confidence_1/1
  IMAPve_g_L0_W/1 -> IMAPve_g_L0_W_convert/1
  IMAPve_g_L0_W_convert/1 -> IMAPve_g_L0_W_1/1
  IMAPve_g_L0_TLC/1 -> IMAPve_g_L0_TLC_convert/1
  IMAPve_g_L0_TLC_convert/1 -> IMAPve_g_L0_TLC_1/1
  IMAPve_d_L0_LC/1 -> IMAPve_d_L0_LC_convert/1
  IMAPve_d_L0_LC_convert/1 -> IMAPve_d_L0_LC_1/1
  IMAPve_g_R0_C0/1 -> IMAPve_g_R0_C0_convert/1
  IMAPve_g_R0_C0_convert/1 -> IMAPve_g_R0_C0_1/1
  IMAPve_g_R0_C1/1 -> IMAPve_g_R0_C1_convert/1
  IMAPve_g_R0_C1_convert/1 -> IMAPve_g_R0_C1_1/1
  IMAPve_g_R0_C2/1 -> IMAPve_g_R0_C2_convert/1
  IMAPve_g_R0_C2_convert/1 -> IMAPve_g_R0_C2_1/1
  IMAPve_g_R0_C3/1 -> IMAPve_g_R0_C3_convert/1
  IMAPve_g_R0_C3_convert/1 -> IMAPve_g_R0_C3_1/1
  IMAPve_g_R0_VR/1 -> IMAPve_g_R0_VR_convert/1
  IMAPve_g_R0_VR_convert/1 -> IMAPve_g_R0_VR_1/1
  IMAPve_d_R0_Q/1 -> IMAPve_d_R0_Q_convert/1
  IMAPve_d_R0_Q_convert/1 -> IMAPve_d_R0_Q_1/1
  IMAPve_d_R0_Type/1 -> IMAPve_d_R0_Type_convert/1
  IMAPve_d_R0_Type_convert/1 -> IMAPve_d_R0_Type_1/1
  IMAPve_g_R0_Confidence/1 -> IMAPve_g_R0_Confidence_convert/1
  IMAPve_g_R0_Confidence_convert/1 -> IMAPve_g_R0_Confidence_1/1
  IMAPve_g_R0_W/1 -> IMAPve_g_R0_W_convert/1
  IMAPve_g_R0_W_convert/1 -> IMAPve_g_R0_W_1/1
  IMAPve_g_R0_TLC/1 -> IMAPve_g_R0_TLC_convert/1
  IMAPve_g_R0_TLC_convert/1 -> IMAPve_g_R0_TLC_1/1
  IMAPve_d_R0_LC/1 -> IMAPve_d_R0_LC_convert/1
  IMAPve_d_R0_LC_convert/1 -> IMAPve_d_R0_LC_1/1
  IMAPve_g_L1_C0/1 -> IMAPve_g_L1_C0_convert/1
  IMAPve_g_L1_C0_convert/1 -> IMAPve_g_L1_C0_1/1
  IMAPve_g_L1_C1/1 -> IMAPve_g_L1_C1_convert/1
  IMAPve_g_L1_C1_convert/1 -> IMAPve_g_L1_C1_1/1
  IMAPve_g_L1_C2/1 -> IMAPve_g_L1_C2_convert/1
  IMAPve_g_L1_C2_convert/1 -> IMAPve_g_L1_C2_1/1
  IMAPve_g_L1_C3/1 -> IMAPve_g_L1_C3_convert/1
  IMAPve_g_L1_C3_convert/1 -> IMAPve_g_L1_C3_1/1
  IMAPve_g_L1_VR/1 -> IMAPve_g_L1_VR_convert/1
  IMAPve_g_L1_VR_convert/1 -> IMAPve_g_L1_VR_1/1
  IMAPve_d_L1_Q/1 -> IMAPve_d_L1_Q_convert/1
  IMAPve_d_L1_Q_convert/1 -> IMAPve_d_L1_Q_1/1
  IMAPve_d_L1_Type/1 -> IMAPve_d_L1_Type_convert/1
  IMAPve_d_L1_Type_convert/1 -> IMAPve_d_L1_Type_1/1
  IMAPve_g_L1_Confidence/1 -> IMAPve_g_L1_Confidence_convert/1
  IMAPve_g_L1_Confidence_convert/1 -> IMAPve_g_L1_Confidence_1/1
  IMAPve_g_L1_W/1 -> IMAPve_g_L1_W_convert/1
  IMAPve_g_L1_W_convert/1 -> IMAPve_g_L1_W_1/1
  IMAPve_g_L1_TLC/1 -> IMAPve_g_L1_TLC_convert/1
  IMAPve_g_L1_TLC_convert/1 -> IMAPve_g_L1_TLC_1/1
  IMAPve_d_L1_LC/1 -> IMAPve_d_L1_LC_convert/1
  IMAPve_d_L1_LC_convert/1 -> IMAPve_d_L1_LC_1/1
  IMAPve_g_R1_C0/1 -> IMAPve_g_R1_C0_convert/1
  IMAPve_g_R1_C0_convert/1 -> IMAPve_g_R1_C0_1/1
  IMAPve_g_R1_C1/1 -> IMAPve_g_R1_C1_convert/1
  IMAPve_g_R1_C1_convert/1 -> IMAPve_g_R1_C1_1/1
  IMAPve_g_R1_C2/1 -> IMAPve_g_R1_C2_convert/1
  IMAPve_g_R1_C2_convert/1 -> IMAPve_g_R1_C2_1/1
  IMAPve_g_R1_C3/1 -> IMAPve_g_R1_C3_convert/1
  IMAPve_g_R1_C3_convert/1 -> IMAPve_g_R1_C3_1/1
  IMAPve_g_R1_VR/1 -> IMAPve_g_R1_VR_convert/1
  IMAPve_g_R1_VR_convert/1 -> IMAPve_g_R1_VR_1/1
  IMAPve_d_R1_Q/1 -> IMAPve_d_R1_Q_convert/1
  IMAPve_d_R1_Q_convert/1 -> IMAPve_d_R1_Q_1/1
  IMAPve_d_R1_Type/1 -> IMAPve_d_R1_Type_convert/1
  IMAPve_d_R1_Type_convert/1 -> IMAPve_d_R1_Type_1/1
  IMAPve_g_R1_Confidence/1 -> IMAPve_g_R1_Confidence_convert/1
  IMAPve_g_R1_Confidence_convert/1 -> IMAPve_g_R1_Confidence_1/1
  IMAPve_g_R1_W/1 -> IMAPve_g_R1_W_convert/1
  IMAPve_g_R1_W_convert/1 -> IMAPve_g_R1_W_1/1
  IMAPve_g_R1_TLC/1 -> IMAPve_g_R1_TLC_convert/1
  IMAPve_g_R1_TLC_convert/1 -> IMAPve_g_R1_TLC_1/1
  IMAPve_d_R1_LC/1 -> IMAPve_d_R1_LC_convert/1
  IMAPve_d_R1_LC_convert/1 -> IMAPve_d_R1_LC_1/1
  IMAPve_g_L0_C0_Back/1 -> IMAPve_g_L0_C0_Back_convert/1
  IMAPve_g_L0_C0_Back_convert/1 -> IMAPve_g_L0_C0_Back_1/1
  IMAPve_g_L0_C1_Back/1 -> IMAPve_g_L0_C1_Back_convert/1
  IMAPve_g_L0_C1_Back_convert/1 -> IMAPve_g_L0_C1_Back_1/1
  IMAPve_g_L0_C2_Back/1 -> IMAPve_g_L0_C2_Back_convert/1
  IMAPve_g_L0_C2_Back_convert/1 -> IMAPve_g_L0_C2_Back_1/1
  IMAPve_g_L0_C3_Back/1 -> IMAPve_g_L0_C3_Back_convert/1
  IMAPve_g_L0_C3_Back_convert/1 -> IMAPve_g_L0_C3_Back_1/1
  IMAPve_g_L0_Range_Back/1 -> IMAPve_g_L0_Range_Back_convert/1
  IMAPve_g_L0_Range_Back_convert/1 -> IMAPve_g_L0_Range_Back_1/1
  IMAPve_g_L0_C0_FR_Pred/1 -> IMAPve_g_L0_C0_FR_Pred_convert/1
  IMAPve_g_L0_C0_FR_Pred_convert/1 -> IMAPve_g_L0_C0_FR_Pred_1/1
  IMAPve_g_L0_C1_FR_Pred/1 -> IMAPve_g_L0_C1_FR_Pred_convert/1
  IMAPve_g_L0_C1_FR_Pred_convert/1 -> IMAPve_g_L0_C1_FR_Pred_1/1
  IMAPve_g_L0_C2_FR_Pred/1 -> IMAPve_g_L0_C2_FR_Pred_convert/1
  IMAPve_g_L0_C2_FR_Pred_convert/1 -> IMAPve_g_L0_C2_FR_Pred_1/1
  IMAPve_g_L0_Range_FR_Pred/1 -> IMAPve_g_L0_Range_FR_Pred_convert/1
  IMAPve_g_L0_Range_FR_Pred_convert/1 -> IMAPve_g_L0_Range_FR_Pred_1/1
  IMAPve_g_R0_C0_Back/1 -> IMAPve_g_R0_C0_Back_convert/1
  IMAPve_g_R0_C0_Back_convert/1 -> IMAPve_g_R0_C0_Back_1/1
  IMAPve_g_R0_C1_Back/1 -> IMAPve_g_R0_C1_Back_convert/1
  IMAPve_g_R0_C1_Back_convert/1 -> IMAPve_g_R0_C1_Back_1/1
  IMAPve_g_R0_C2_Back/1 -> IMAPve_g_R0_C2_Back_convert/1
  IMAPve_g_R0_C2_Back_convert/1 -> IMAPve_g_R0_C2_Back_1/1
  IMAPve_g_R0_C3_Back/1 -> IMAPve_g_R0_C3_Back_convert/1
  IMAPve_g_R0_C3_Back_convert/1 -> IMAPve_g_R0_C3_Back_1/1
  IMAPve_g_R0_Range_Back/1 -> IMAPve_g_R0_Range_Back_convert/1
  IMAPve_g_R0_Range_Back_convert/1 -> IMAPve_g_R0_Range_Back_1/1
  IMAPve_g_R0_C0_FR_Pred/1 -> IMAPve_g_R0_C0_FR_Pred_convert/1
  IMAPve_g_R0_C0_FR_Pred_convert/1 -> IMAPve_g_R0_C0_FR_Pred_1/1
  IMAPve_g_R0_C1_FR_Pred/1 -> IMAPve_g_R0_C1_FR_Pred_convert/1
  IMAPve_g_R0_C1_FR_Pred_convert/1 -> IMAPve_g_R0_C1_FR_Pred_1/1
  IMAPve_g_R0_C2_FR_Pred/1 -> IMAPve_g_R0_C2_FR_Pred_convert/1
  IMAPve_g_R0_C2_FR_Pred_convert/1 -> IMAPve_g_R0_C2_FR_Pred_1/1
  IMAPve_g_R0_Range_FR_Pred/1 -> IMAPve_g_R0_Range_FR_Pred_convert/1
  IMAPve_g_R0_Range_FR_Pred_convert/1 -> IMAPve_g_R0_Range_FR_Pred_1/1
  IMAPve_g_L1_C0_Back/1 -> IMAPve_g_L1_C0_Back_convert/1
  IMAPve_g_L1_C0_Back_convert/1 -> IMAPve_g_L1_C0_Back_1/1
  IMAPve_g_L1_C1_Back/1 -> IMAPve_g_L1_C1_Back_convert/1
  IMAPve_g_L1_C1_Back_convert/1 -> IMAPve_g_L1_C1_Back_1/1
  IMAPve_g_L1_C2_Back/1 -> IMAPve_g_L1_C2_Back_convert/1
  IMAPve_g_L1_C2_Back_convert/1 -> IMAPve_g_L1_C2_Back_1/1
  IMAPve_g_L1_C3_Back/1 -> IMAPve_g_L1_C3_Back_convert/1
  IMAPve_g_L1_C3_Back_convert/1 -> IMAPve_g_L1_C3_Back_1/1
  IMAPve_g_L1_Range_Back/1 -> IMAPve_g_L1_Range_Back_convert/1
  IMAPve_g_L1_Range_Back_convert/1 -> IMAPve_g_L1_Range_Back_1/1
  IMAPve_g_L1_C0_FR_Pred/1 -> IMAPve_g_L1_C0_FR_Pred_convert/1
  IMAPve_g_L1_C0_FR_Pred_convert/1 -> IMAPve_g_L1_C0_FR_Pred_1/1
  IMAPve_g_L1_C1_FR_Pred/1 -> IMAPve_g_L1_C1_FR_Pred_convert/1
  IMAPve_g_L1_C1_FR_Pred_convert/1 -> IMAPve_g_L1_C1_FR_Pred_1/1
  IMAPve_g_L1_C2_FR_Pred/1 -> IMAPve_g_L1_C2_FR_Pred_convert/1
  IMAPve_g_L1_C2_FR_Pred_convert/1 -> IMAPve_g_L1_C2_FR_Pred_1/1
  IMAPve_g_L1_Range_FR_Pred/1 -> IMAPve_g_L1_Range_FR_Pred_convert/1
  IMAPve_g_L1_Range_FR_Pred_convert/1 -> IMAPve_g_L1_Range_FR_Pred_1/1
  IMAPve_g_R1_C0_Back/1 -> IMAPve_g_R1_C0_Back_convert/1
  IMAPve_g_R1_C0_Back_convert/1 -> IMAPve_g_R1_C0_Back_1/1
  IMAPve_g_R1_C1_Back/1 -> IMAPve_g_R1_C1_Back_convert/1
  IMAPve_g_R1_C1_Back_convert/1 -> IMAPve_g_R1_C1_Back_1/1
  IMAPve_g_R1_C2_Back/1 -> IMAPve_g_R1_C2_Back_convert/1
  IMAPve_g_R1_C2_Back_convert/1 -> IMAPve_g_R1_C2_Back_1/1
  IMAPve_g_R1_C3_Back/1 -> IMAPve_g_R1_C3_Back_convert/1
  IMAPve_g_R1_C3_Back_convert/1 -> IMAPve_g_R1_C3_Back_1/1
  IMAPve_g_R1_Range_Back/1 -> IMAPve_g_R1_Range_Back_convert/1
  IMAPve_g_R1_Range_Back_convert/1 -> IMAPve_g_R1_Range_Back_1/1
  IMAPve_g_R1_C0_FR_Pred/1 -> IMAPve_g_R1_C0_FR_Pred_convert/1
  IMAPve_g_R1_C0_FR_Pred_convert/1 -> IMAPve_g_R1_C0_FR_Pred_1/1
  IMAPve_g_R1_C1_FR_Pred/1 -> IMAPve_g_R1_C1_FR_Pred_convert/1
  IMAPve_g_R1_C1_FR_Pred_convert/1 -> IMAPve_g_R1_C1_FR_Pred_1/1
  IMAPve_g_R1_C2_FR_Pred/1 -> IMAPve_g_R1_C2_FR_Pred_convert/1
  IMAPve_g_R1_C2_FR_Pred_convert/1 -> IMAPve_g_R1_C2_FR_Pred_1/1
  IMAPve_g_R1_Range_FR_Pred/1 -> IMAPve_g_R1_Range_FR_Pred_convert/1
  IMAPve_g_R1_Range_FR_Pred_convert/1 -> IMAPve_g_R1_Range_FR_Pred_1/1
  IMAPve_d_Sign_ISA_Value/1 -> IMAPve_d_Sign_ISA_Value_convert/1
  IMAPve_d_Sign_ISA_Value_convert/1 -> IMAPve_d_Sign_ISA_Value_1/1
  IMAPve_d_TSR_Sign_Type/1 -> IMAPve_d_TSR_Sign_Type_convert/1
  IMAPve_d_TSR_Sign_Type_convert/1 -> IMAPve_d_TSR_Sign_Type_1/1
  IMAPve_d_Camera_Signal_Fault/1 -> IMAPve_d_Camera_Signal_Fault_convert/1
  IMAPve_d_Camera_Signal_Fault_convert/1 -> IMAPve_d_Camera_Signal_Fault_1/1
  IMAPve_d_Radar_Status/1 -> IMAPve_d_Radar_Status_convert/1
  IMAPve_d_Radar_Status_convert/1 -> IMAPve_d_Radar_Status_1/1
  IMAPve_d_Camera_Status/1 -> IMAPve_d_Camera_Status_convert/1
  IMAPve_d_Camera_Status_convert/1 -> IMAPve_d_Camera_Status_1/1
  IMAPva_d_obj_id/1 -> IMAPva_d_obj_id_convert/1  "IMAPva_d_obj_id"
  IMAPva_g_obj_con/1 -> IMAPva_g_obj_con_convert/1  "IMAPva_g_obj_con"
  IMAPva_d_obj_MotionStatus/1 -> IMAPva_d_obj_MotionStatus_convert/1  "IMAPva_d_obj_MotionStatus"
  Data Type Conversion4/1 -> ICARva_d_obj_Num/1  "<signal1>"
  Data Type Conversion6/1 -> ICARva_d_obj_id/1
  Data Type Conversion14/1 -> ICARva_g_obj_pos_x/1
  Data Type Conversion15/1 -> ICARva_g_obj_pos_y/1
  Data Type Conversion16/1 -> ICARva_g_obj_vel_x/1
  Data Type Conversion17/1 -> ICARva_g_obj_vel_y/1
  Data Type Conversion18/1 -> ICARva_g_obj_acc_x/1
  Data Type Conversion19/1 -> ICARva_g_obj_acc_y/1
  Data Type Conversion20/1 -> ICARva_g_obj_pos_var_x/1
  Data Type Conversion21/1 -> ICARva_g_obj_pos_var_y/1
  Data Type Conversion22/1 -> ICARva_g_obj_pos_var_xy/1
  Data Type Conversion23/1 -> ICARva_g_obj_vel_var_x/1
  Data Type Conversion24/1 -> ICARva_g_obj_vel_var_y/1
  Data Type Conversion25/1 -> ICARva_g_obj_vel_var_xy/1
  Data Type Conversion26/1 -> ICARva_g_obj_width/1
  Data Type Conversion7/1 -> ICARva_d_obj_fusion_type/1
  Data Type Conversion8/1 -> ICARva_d_obj_class/1
  Data Type Conversion9/1 -> ICARva_d_obj_lane/1
  Data Type Conversion10/1 -> ICARva_d_obj_status/1
  Data Type Conversion2/1 -> ICARva_g_obj_con/1
  Data Type Conversion3/1 -> ICARva_d_obj_TurnLi/1
  Data Type Conversion12/1 -> ICARva_d_obj_BrkLi/1
  Data Type Conversion13/1 -> ICARva_d_obj_MtnStat/1
  MATLAB Function/1(y) -> Data Type Conversion/1
  Data Type Conversion/1 -> ICARva_g_ObjVelVarXYPre/1, ICARva_g_ObjVelVarYPre/1, ICARva_g_ObjVelVarXPre/1, ICARva_g_ObjVelYPre/1, ICARva_g_ObjVelXPre/1, ICARva_g_ObjVarXYPre/1, ICARva_g_ObjVarYPre/1, ICARva_g_ObjVarXPre/1, ICARva_g_ObjYPre/1, ICARva_g_ObjXPre/1
  Data Type Conversion1/1 -> ICARve_d_SignalTStamp/1
  Constant/1 -> Data Type Conversion1/1
  Data Type Conversion27/1 -> ICARva_d_obj_length/1
  Data Type Conversion11/1 -> ICARva_d_obj_age/1
  Data Type Conversion5/1 -> ICARve_d_obj_cam_asso_id/1  "<signal1>"
  MATLAB Function1/1(y) -> Data Type Conversion4/1
  Constant1/1 -> Data Type Conversion5/1
  MATLAB Function3/1(y) -> Data Type Conversion6/1
  MATLAB Function4/1(y) -> Data Type Conversion7/1
  MATLAB Function5/1(y) -> Data Type Conversion8/1
  MATLAB Function6/1(y) -> Data Type Conversion9/1
  MATLAB Function7/1(y) -> Data Type Conversion10/1
  MATLAB Function8/1(y) -> Data Type Conversion11/1
  MATLAB Function9/1(y) -> Data Type Conversion3/1
  MATLAB Function10/1(y) -> Data Type Conversion12/1
  MATLAB Function11/1(y) -> Data Type Conversion13/1
  MATLAB Function12/1(y) -> Data Type Conversion14/1
  MATLAB Function13/1(y) -> Data Type Conversion15/1
  MATLAB Function14/1(y) -> Data Type Conversion16/1
  MATLAB Function15/1(y) -> Data Type Conversion17/1
  MATLAB Function16/1(y) -> Data Type Conversion18/1
  MATLAB Function17/1(y) -> Data Type Conversion19/1
  MATLAB Function18/1(y) -> Data Type Conversion20/1
  MATLAB Function19/1(y) -> Data Type Conversion21/1
  MATLAB Function20/1(y) -> Data Type Conversion22/1
  MATLAB Function21/1(y) -> Data Type Conversion23/1
  MATLAB Function22/1(y) -> Data Type Conversion24/1
  MATLAB Function23/1(y) -> Data Type Conversion25/1
  MATLAB Function24/1(y) -> Data Type Conversion26/1
  MATLAB Function25/1(y) -> Data Type Conversion27/1
  MATLAB Function26/1(y) -> Data Type Conversion2/1
